simulink model "model"  (R2014a)
(part 8 of 8)

  T_26367884_110000_/LConn1 -- _CN_26391332_110000_CN_26367884_110000/RConn1
  T_26367884_110000_/LConn2 -- _CN_26391332_110000_CN_26367884_110000/RConn2
  _CN_26391332_110000_CN_26367884_110000/RConn3 -- T_26367884_110000_/LConn3 -- bus192/LConn1
  T_197245741_110000_/LConn1 -- _CN_197245741_110000_CN_128571463_110000/RConn1
  T_197245741_110000_/LConn2 -- _CN_197245741_110000_CN_128571463_110000/RConn2
  _CN_197245741_110000_CN_128571463_110000/RConn3 -- T_197245741_110000_/LConn3 -- bus193/LConn1
  _CN_117383986_110000_CN_153576520_110000/RConn1 -- T_153576520_110000_/LConn1 -- _CN_153576520_110000_CN_148596527_110000/RConn1
  _CN_117383986_110000_CN_153576520_110000/RConn2 -- T_153576520_110000_/LConn2 -- _CN_153576520_110000_CN_148596527_110000/RConn2
  _CN_117383986_110000_CN_153576520_110000/RConn3 -- T_153576520_110000_/LConn3 -- _CN_153576520_110000_CN_148596527_110000/RConn3 -- bus194/LConn1
  _CN_47317827_110000_CN_169899622_110000/LConn1 -- T_47317827_400000;110000_Keminmaan_sähköasema/RConn1 -- _CN_47317827_110000_CN_118766661_110000/RConn1 -- L_47317827/LConn1
  _CN_47317827_110000_CN_169899622_110000/LConn2 -- T_47317827_400000;110000_Keminmaan_sähköasema/RConn2 -- _CN_47317827_110000_CN_118766661_110000/RConn2 -- L_47317827/LConn2
  _CN_47317827_110000_CN_169899622_110000/LConn3 -- T_47317827_400000;110000_Keminmaan_sähköasema/RConn3 -- _CN_47317827_110000_CN_118766661_110000/RConn3 -- L_47317827/LConn3 -- bus195/LConn1
  _CN_47317827_110000_CN_169899622_110000/RConn1 -- T_169899622_220000;110000_/LConn1 -- _CN_169899622_110000_CN_169899620_20000/RConn1
  _CN_47317827_110000_CN_169899622_110000/RConn2 -- T_169899622_220000;110000_/LConn2 -- _CN_169899622_110000_CN_169899620_20000/RConn2
  _CN_47317827_110000_CN_169899622_110000/RConn3 -- T_169899622_220000;110000_/LConn3 -- _CN_169899622_110000_CN_169899620_20000/RConn3 -- bus196/LConn1
  _CN_137112425_110000_CN_132652863_110000/LConn1 -- T_137112425_110000_/LConn1 -- _CN_137112425_110000_CN_136355274_110000/LConn1
  _CN_137112425_110000_CN_132652863_110000/LConn2 -- T_137112425_110000_/LConn2 -- _CN_137112425_110000_CN_136355274_110000/LConn2
  _CN_137112425_110000_CN_132652863_110000/LConn3 -- T_137112425_110000_/LConn3 -- _CN_137112425_110000_CN_136355274_110000/LConn3 -- bus197/LConn1
  T_132652863__/LConn1 -- _CN_137112425_110000_CN_132652863_110000/RConn1
  T_132652863__/LConn2 -- _CN_137112425_110000_CN_132652863_110000/RConn2
  _CN_137112425_110000_CN_132652863_110000/RConn3 -- T_132652863__/LConn3 -- bus198/LConn1
  _CN_137112425_110000_CN_136355274_110000/RConn1 -- T_136355274_110000_/LConn1 -- _CN_136355274_110000_CN_136361669_110000/LConn1
  _CN_137112425_110000_CN_136355274_110000/RConn2 -- T_136355274_110000_/LConn2 -- _CN_136355274_110000_CN_136361669_110000/LConn2
  _CN_137112425_110000_CN_136355274_110000/RConn3 -- T_136355274_110000_/LConn3 -- _CN_136355274_110000_CN_136361669_110000/LConn3 -- bus199/LConn1
  T_211471223_110000_/LConn1 -- _CN_211471223_110000_CN_98613134_110000/LConn1
  T_211471223_110000_/LConn2 -- _CN_211471223_110000_CN_98613134_110000/LConn2
  _CN_211471223_110000_CN_98613134_110000/LConn3 -- T_211471223_110000_/LConn3 -- bus200/LConn1
  _CN_211471223_110000_CN_98613134_110000/RConn1 -- T_98613134_400000;110000_/RConn1 -- _CN_26501426_110000_CN_98613134_110000/RConn1 -- L_98613134/LConn1
  _CN_211471223_110000_CN_98613134_110000/RConn2 -- T_98613134_400000;110000_/RConn2 -- _CN_26501426_110000_CN_98613134_110000/RConn2 -- L_98613134/LConn2
  _CN_211471223_110000_CN_98613134_110000/RConn3 -- T_98613134_400000;110000_/RConn3 -- _CN_26501426_110000_CN_98613134_110000/RConn3 -- L_98613134/LConn3 -- bus201/LConn1
  T_129112047_110000_/LConn1 -- _CN_128463750_110000_CN_129112047_110000/RConn1
  T_129112047_110000_/LConn2 -- _CN_128463750_110000_CN_129112047_110000/RConn2
  _CN_128463750_110000_CN_129112047_110000/RConn3 -- T_129112047_110000_/LConn3 -- bus202/LConn1
  T_155899286_110000_/LConn1 -- _CN_128463750_110000_CN_155899286_110000/RConn1
  T_155899286_110000_/LConn2 -- _CN_128463750_110000_CN_155899286_110000/RConn2
  _CN_128463750_110000_CN_155899286_110000/RConn3 -- T_155899286_110000_/LConn3 -- bus203/LConn1
  T_94667682_110000_/LConn1 -- _CN_94667682_110000_CN_95184246_110000/LConn1
  T_94667682_110000_/LConn2 -- _CN_94667682_110000_CN_95184246_110000/LConn2
  _CN_94667682_110000_CN_95184246_110000/LConn3 -- T_94667682_110000_/LConn3 -- bus204/LConn1
  T_95184246_110000_/LConn1 -- _CN_94667682_110000_CN_95184246_110000/RConn1
  T_95184246_110000_/LConn2 -- _CN_94667682_110000_CN_95184246_110000/RConn2
  _CN_94667682_110000_CN_95184246_110000/RConn3 -- T_95184246_110000_/LConn3 -- bus205/LConn1
  T_142846911__/LConn1 -- _CN_142846911_110000_CN_142846913_110000/RConn1
  T_142846911__/LConn2 -- _CN_142846911_110000_CN_142846913_110000/RConn2
  _CN_142846911_110000_CN_142846913_110000/RConn3 -- T_142846911__/LConn3 -- bus206/LConn1
  T_200166363__/LConn1 -- _CN_200166363_110000_CN_173431812_110000/LConn1
  T_200166363__/LConn2 -- _CN_200166363_110000_CN_173431812_110000/LConn2
  _CN_200166363_110000_CN_173431812_110000/LConn3 -- T_200166363__/LConn3 -- bus207/LConn1
  _CN_200166363_110000_CN_173431812_110000/RConn1 -- T_173431812_220000;110000_/LConn1 -- _CN_173431812_110000_CN_285201507_110000/LConn1
  _CN_200166363_110000_CN_173431812_110000/RConn2 -- T_173431812_220000;110000_/LConn2 -- _CN_173431812_110000_CN_285201507_110000/LConn2
  _CN_200166363_110000_CN_173431812_110000/RConn3 -- T_173431812_220000;110000_/LConn3 -- _CN_173431812_110000_CN_285201507_110000/LConn3 -- bus208/LConn1
  _CN_400589797_110000_CN_61960767_110000/LConn1 -- T_400589797_110000_/LConn1 -- _CN_400589797_110000_CN_400588215_110000/LConn1 -- _CN_400589797_110000_CN_92656655_110000/LConn1 -- _CN_400589797_110000_CN_174266079_110000/LConn1
  _CN_400589797_110000_CN_61960767_110000/LConn2 -- T_400589797_110000_/LConn2 -- _CN_400589797_110000_CN_400588215_110000/LConn2 -- _CN_400589797_110000_CN_92656655_110000/LConn2 -- _CN_400589797_110000_CN_174266079_110000/LConn2
  _CN_400589797_110000_CN_61960767_110000/LConn3 -- T_400589797_110000_/LConn3 -- _CN_400589797_110000_CN_400588215_110000/LConn3 -- _CN_400589797_110000_CN_92656655_110000/LConn3 -- _CN_400589797_110000_CN_174266079_110000/LConn3 -- bus209/LConn1
  G_61960767_/RConn1 -- _CN_400589797_110000_CN_61960767_110000/RConn1
  G_61960767_/RConn2 -- _CN_400589797_110000_CN_61960767_110000/RConn2
  _CN_400589797_110000_CN_61960767_110000/RConn3 -- G_61960767_/RConn3 -- bus210/LConn1
  _CN_400589797_110000_CN_400588215_110000/RConn1 -- T_400588215_110000_/LConn1 -- _CN_400588215_110000_CN_400588216_110000/RConn1
  _CN_400589797_110000_CN_400588215_110000/RConn2 -- T_400588215_110000_/LConn2 -- _CN_400588215_110000_CN_400588216_110000/RConn2
  _CN_400589797_110000_CN_400588215_110000/RConn3 -- T_400588215_110000_/LConn3 -- _CN_400588215_110000_CN_400588216_110000/RConn3 -- bus211/LConn1
  _CN_400589797_110000_CN_92656655_110000/RConn1 -- T_92656655_110000_/LConn1 -- _CN_363802508_110000_CN_92656655_110000/LConn1
  _CN_400589797_110000_CN_92656655_110000/RConn2 -- T_92656655_110000_/LConn2 -- _CN_363802508_110000_CN_92656655_110000/LConn2
  _CN_400589797_110000_CN_92656655_110000/RConn3 -- T_92656655_110000_/LConn3 -- _CN_363802508_110000_CN_92656655_110000/LConn3 -- bus212/LConn1
  T_174266079__/LConn1 -- _CN_400589797_110000_CN_174266079_110000/RConn1
  T_174266079__/LConn2 -- _CN_400589797_110000_CN_174266079_110000/RConn2
  _CN_400589797_110000_CN_174266079_110000/RConn3 -- T_174266079__/LConn3 -- bus213/LConn1
  T_363802508_110000_/LConn1 -- _CN_363802508_110000_CN_92656655_110000/RConn1
  T_363802508_110000_/LConn2 -- _CN_363802508_110000_CN_92656655_110000/RConn2
  _CN_363802508_110000_CN_92656655_110000/RConn3 -- T_363802508_110000_/LConn3 -- bus214/LConn1
  _CN_96660466_110000_CN_98393115_110000/LConn1 -- T_96660466_400000;110000_/RConn1 -- L_96660466/LConn1
  _CN_96660466_110000_CN_98393115_110000/LConn2 -- T_96660466_400000;110000_/RConn2 -- L_96660466/LConn2
  _CN_96660466_110000_CN_98393115_110000/LConn3 -- T_96660466_400000;110000_/RConn3 -- L_96660466/LConn3 -- bus215/LConn1
  T_98393115_110000_/LConn1 -- _CN_96660466_110000_CN_98393115_110000/RConn1
  T_98393115_110000_/LConn2 -- _CN_96660466_110000_CN_98393115_110000/RConn2
  _CN_96660466_110000_CN_98393115_110000/RConn3 -- T_98393115_110000_/LConn3 -- bus216/LConn1
  T_391142388_220000;110000_/LConn1 -- _CN_391142388_110000_CN_391142037_110000/LConn1
  T_391142388_220000;110000_/LConn2 -- _CN_391142388_110000_CN_391142037_110000/LConn2
  _CN_391142388_110000_CN_391142037_110000/LConn3 -- T_391142388_220000;110000_/LConn3 -- bus217/LConn1
  T_391142037_110000_/LConn1 -- _CN_391142388_110000_CN_391142037_110000/RConn1
  T_391142037_110000_/LConn2 -- _CN_391142388_110000_CN_391142037_110000/RConn2
  _CN_391142388_110000_CN_391142037_110000/RConn3 -- T_391142037_110000_/LConn3 -- bus218/LConn1
  _CN_173431802_110000_CN_122703556_110000/LConn1 -- T_173431802_400000;110000_/RConn1 -- L_173431802/LConn1
  _CN_173431802_110000_CN_122703556_110000/LConn2 -- T_173431802_400000;110000_/RConn2 -- L_173431802/LConn2
  _CN_173431802_110000_CN_122703556_110000/LConn3 -- T_173431802_400000;110000_/RConn3 -- L_173431802/LConn3 -- bus219/LConn1
  T_122703556__/LConn1 -- _CN_173431802_110000_CN_122703556_110000/RConn1
  T_122703556__/LConn2 -- _CN_173431802_110000_CN_122703556_110000/RConn2
  _CN_173431802_110000_CN_122703556_110000/RConn3 -- T_122703556__/LConn3 -- bus220/LConn1
  T_285201507__/LConn1 -- _CN_173431812_110000_CN_285201507_110000/RConn1
  T_285201507__/LConn2 -- _CN_173431812_110000_CN_285201507_110000/RConn2
  _CN_173431812_110000_CN_285201507_110000/RConn3 -- T_285201507__/LConn3 -- bus221/LConn1
  _CN_235817994_110000_CN_89956002_110000/LConn1 -- T_235817994_110000_/LConn1 -- _CN_235817994_110000_CN_345672987_110000/LConn1 -- _CN_235817994_110000_CN_88020737_110000/LConn1 -- _CN_235817994_110000_CN_88020687_110000/LConn1
  _CN_235817994_110000_CN_89956002_110000/LConn2 -- T_235817994_110000_/LConn2 -- _CN_235817994_110000_CN_345672987_110000/LConn2 -- _CN_235817994_110000_CN_88020737_110000/LConn2 -- _CN_235817994_110000_CN_88020687_110000/LConn2
  _CN_235817994_110000_CN_89956002_110000/LConn3 -- T_235817994_110000_/LConn3 -- _CN_235817994_110000_CN_345672987_110000/LConn3 -- bus222/LConn1 -- _CN_235817994_110000_CN_88020737_110000/LConn3 -- _CN_235817994_110000_CN_88020687_110000/LConn3
  T_89956002_110000_/LConn1 -- _CN_235817994_110000_CN_89956002_110000/RConn1
  T_89956002_110000_/LConn2 -- _CN_235817994_110000_CN_89956002_110000/RConn2
  _CN_235817994_110000_CN_89956002_110000/RConn3 -- T_89956002_110000_/LConn3 -- bus223/LConn1
  T_88020737_110000_/LConn1 -- _CN_235817994_110000_CN_88020737_110000/RConn1
  T_88020737_110000_/LConn2 -- _CN_235817994_110000_CN_88020737_110000/RConn2
  _CN_235817994_110000_CN_88020737_110000/RConn3 -- T_88020737_110000_/LConn3 -- bus224/LConn1
  T_88020687_110000_/LConn1 -- _CN_235817994_110000_CN_88020687_110000/RConn1
  T_88020687_110000_/LConn2 -- _CN_235817994_110000_CN_88020687_110000/RConn2
  _CN_235817994_110000_CN_88020687_110000/RConn3 -- T_88020687_110000_/LConn3 -- bus225/LConn1
  _CN_235817994_110000_CN_345672987_110000/RConn1 -- T_345672987_110000_/LConn1 -- _CN_345672987_110000_CN_348349199_110000/LConn1
  _CN_235817994_110000_CN_345672987_110000/RConn2 -- T_345672987_110000_/LConn2 -- _CN_345672987_110000_CN_348349199_110000/LConn2
  _CN_235817994_110000_CN_345672987_110000/RConn3 -- T_345672987_110000_/LConn3 -- _CN_345672987_110000_CN_348349199_110000/LConn3 -- bus226/LConn1
  T_30483473__/LConn1 -- _CN_30483473_110000_CN_40101584_110000/RConn1
  T_30483473__/LConn2 -- _CN_30483473_110000_CN_40101584_110000/RConn2
  _CN_30483473_110000_CN_40101584_110000/RConn3 -- T_30483473__/LConn3 -- bus227/LConn1
  _CN_28785740_110000_CN_28820749_110000/RConn1 -- T_28820749_400000;110000_Länsisalmen_sähköasema/RConn1 -- L_28820749/LConn1
  _CN_28785740_110000_CN_28820749_110000/RConn2 -- T_28820749_400000;110000_Länsisalmen_sähköasema/RConn2 -- L_28820749/LConn2
  _CN_28785740_110000_CN_28820749_110000/RConn3 -- T_28820749_400000;110000_Länsisalmen_sähköasema/RConn3 -- L_28820749/LConn3 -- bus228/LConn1
  T_218734234__/LConn1 -- _CN_32910454_110000_CN_218734234_110000/RConn1
  T_218734234__/LConn2 -- _CN_32910454_110000_CN_218734234_110000/RConn2
  _CN_32910454_110000_CN_218734234_110000/RConn3 -- T_218734234__/LConn3 -- bus229/LConn1
  T_167705754_110000_/LConn1 -- _CN_32910454_110000_CN_167705754_110000/RConn1
  T_167705754_110000_/LConn2 -- _CN_32910454_110000_CN_167705754_110000/RConn2
  _CN_32910454_110000_CN_167705754_110000/RConn3 -- T_167705754_110000_/LConn3 -- bus230/LConn1
  T_122838157_110000_/LConn1 -- _CN_122838157_110000_CN_140227959_110000/LConn1
  T_122838157_110000_/LConn2 -- _CN_122838157_110000_CN_140227959_110000/LConn2
  _CN_122838157_110000_CN_140227959_110000/LConn3 -- T_122838157_110000_/LConn3 -- bus231/LConn1
  T_140227959_110000_/LConn1 -- _CN_122838157_110000_CN_140227959_110000/RConn1
  T_140227959_110000_/LConn2 -- _CN_122838157_110000_CN_140227959_110000/RConn2
  _CN_122838157_110000_CN_140227959_110000/RConn3 -- T_140227959_110000_/LConn3 -- bus232/LConn1
  T_167862173__/LConn1 -- _CN_98561229_110000_CN_167862173_110000/RConn1
  T_167862173__/LConn2 -- _CN_98561229_110000_CN_167862173_110000/RConn2
  _CN_98561229_110000_CN_167862173_110000/RConn3 -- T_167862173__/LConn3 -- bus233/LConn1
  T_345672928__/LConn1 -- _CN_345672928_110000_CN_40101584_110000/RConn1
  T_345672928__/LConn2 -- _CN_345672928_110000_CN_40101584_110000/RConn2
  _CN_345672928_110000_CN_40101584_110000/RConn3 -- T_345672928__/LConn3 -- bus234/LConn1
  _CN_348003562_110000_CN_238900636_110000/RConn1 -- T_348003562_400000;110000_/RConn1 -- _CN_348003562_110000_CN_219227505_110000/RConn1 -- L_348003562/LConn1
  _CN_348003562_110000_CN_238900636_110000/RConn2 -- T_348003562_400000;110000_/RConn2 -- _CN_348003562_110000_CN_219227505_110000/RConn2 -- L_348003562/LConn2
  _CN_348003562_110000_CN_238900636_110000/RConn3 -- T_348003562_400000;110000_/RConn3 -- _CN_348003562_110000_CN_219227505_110000/RConn3 -- L_348003562/LConn3 -- bus235/LConn1
  T_348349199_110000_/LConn1 -- _CN_345672987_110000_CN_348349199_110000/RConn1
  T_348349199_110000_/LConn2 -- _CN_345672987_110000_CN_348349199_110000/RConn2
  _CN_345672987_110000_CN_348349199_110000/RConn3 -- T_348349199_110000_/LConn3 -- bus236/LConn1
  T_162950429_110000_/LConn1 -- _CN_162950429_110000_CN_162690719_110000/LConn1
  T_162950429_110000_/LConn2 -- _CN_162950429_110000_CN_162690719_110000/LConn2
  _CN_162950429_110000_CN_162690719_110000/LConn3 -- T_162950429_110000_/LConn3 -- bus237/LConn1
  T_162690719_110000_/LConn1 -- _CN_162950429_110000_CN_162690719_110000/RConn1
  T_162690719_110000_/LConn2 -- _CN_162950429_110000_CN_162690719_110000/RConn2
  _CN_162950429_110000_CN_162690719_110000/RConn3 -- T_162690719_110000_/LConn3 -- bus238/LConn1
  T_252609822_110000_/LConn1 -- _CN_252609822_110000_CN_150204241_110000/RConn1
  T_252609822_110000_/LConn2 -- _CN_252609822_110000_CN_150204241_110000/RConn2
  _CN_252609822_110000_CN_150204241_110000/RConn3 -- T_252609822_110000_/LConn3 -- bus239/LConn1
  T_158219552_110000_/LConn1 -- _CN_158219552_110000_CN_158031219_110000/RConn1
  T_158219552_110000_/LConn2 -- _CN_158219552_110000_CN_158031219_110000/RConn2
  _CN_158219552_110000_CN_158031219_110000/RConn3 -- T_158219552_110000_/LConn3 -- bus240/LConn1
  T_149818659_110000_/LConn1 -- _CN_149818658_110000_CN_149818659_110000/RConn1
  T_149818659_110000_/LConn2 -- _CN_149818658_110000_CN_149818659_110000/RConn2
  _CN_149818658_110000_CN_149818659_110000/RConn3 -- T_149818659_110000_/LConn3 -- bus241/LConn1
  T_165373253_110000_/LConn1 -- _CN_165373253_110000_CN_154863454_110000/RConn1
  T_165373253_110000_/LConn2 -- _CN_165373253_110000_CN_154863454_110000/RConn2
  _CN_165373253_110000_CN_154863454_110000/RConn3 -- T_165373253_110000_/LConn3 -- bus242/LConn1
  T_130069830__/LConn1 -- _CN_130069830_110000_CN_130069831_110000/LConn1
  T_130069830__/LConn2 -- _CN_130069830_110000_CN_130069831_110000/LConn2
  _CN_130069830_110000_CN_130069831_110000/LConn3 -- T_130069830__/LConn3 -- bus243/LConn1
  T_130069831_110000_/LConn1 -- _CN_130069830_110000_CN_130069831_110000/RConn1
  T_130069831_110000_/LConn2 -- _CN_130069830_110000_CN_130069831_110000/RConn2
  _CN_130069830_110000_CN_130069831_110000/RConn3 -- T_130069831_110000_/LConn3 -- bus244/LConn1
  _CN_130069833_110000_CN_130069838_110000/RConn1 -- T_130069833_110000_/LConn1 -- _CN_130069833_110000_CN_136068907_110000/RConn1
  _CN_130069833_110000_CN_130069838_110000/RConn2 -- T_130069833_110000_/LConn2 -- _CN_130069833_110000_CN_136068907_110000/RConn2
  _CN_130069833_110000_CN_130069838_110000/RConn3 -- T_130069833_110000_/LConn3 -- _CN_130069833_110000_CN_136068907_110000/RConn3 -- bus245/LConn1
  _CN_159532385_110000_CN_108980081_110000/RConn1 -- T_159532385_400000;110000_/RConn1 -- L_159532385/LConn1
  _CN_159532385_110000_CN_108980081_110000/RConn2 -- T_159532385_400000;110000_/RConn2 -- L_159532385/LConn2
  _CN_159532385_110000_CN_108980081_110000/RConn3 -- T_159532385_400000;110000_/RConn3 -- L_159532385/LConn3 -- bus246/LConn1
  T_147699112__/LConn1 -- _CN_147699112_110000_CN_147699118_110000/LConn1
  T_147699112__/LConn2 -- _CN_147699112_110000_CN_147699118_110000/LConn2
  _CN_147699112_110000_CN_147699118_110000/LConn3 -- T_147699112__/LConn3 -- bus247/LConn1
  T_147699118_110000_/LConn1 -- _CN_147699112_110000_CN_147699118_110000/RConn1
  T_147699118_110000_/LConn2 -- _CN_147699112_110000_CN_147699118_110000/RConn2
  _CN_147699112_110000_CN_147699118_110000/RConn3 -- T_147699118_110000_/LConn3 -- bus248/LConn1
  _CN_98735006_110000_CN_400584163_110000/RConn1 -- T_98735006_400000;110000_/RConn1 -- L_98735006/LConn1
  _CN_98735006_110000_CN_400584163_110000/RConn2 -- T_98735006_400000;110000_/RConn2 -- L_98735006/LConn2
  _CN_98735006_110000_CN_400584163_110000/RConn3 -- T_98735006_400000;110000_/RConn3 -- L_98735006/LConn3 -- bus249/LConn1
  T_178234889_110000_/LConn1 -- _CN_26619335_110000_CN_178234889_110000/RConn1
  T_178234889_110000_/LConn2 -- _CN_26619335_110000_CN_178234889_110000/RConn2
  _CN_26619335_110000_CN_178234889_110000/RConn3 -- T_178234889_110000_/LConn3 -- bus250/LConn1
  T_178234890_110000_/LConn1 -- _CN_26619335_110000_CN_178234890_110000/RConn1
  T_178234890_110000_/LConn2 -- _CN_26619335_110000_CN_178234890_110000/RConn2
  _CN_26619335_110000_CN_178234890_110000/RConn3 -- T_178234890_110000_/LConn3 -- bus251/LConn1
  _CN_136355274_110000_CN_136361669_110000/RConn1 -- T_136361669_110000_/LConn1 -- _CN_136361666_110000_CN_136361669_110000/LConn1
  _CN_136355274_110000_CN_136361669_110000/RConn2 -- T_136361669_110000_/LConn2 -- _CN_136361666_110000_CN_136361669_110000/LConn2
  _CN_136355274_110000_CN_136361669_110000/RConn3 -- T_136361669_110000_/LConn3 -- _CN_136361666_110000_CN_136361669_110000/LConn3 -- bus252/LConn1
  T_159172094_110000_/LConn1 -- _CN_159172094_110000_CN_167040166_110000/RConn1
  T_159172094_110000_/LConn2 -- _CN_159172094_110000_CN_167040166_110000/RConn2
  _CN_159172094_110000_CN_167040166_110000/RConn3 -- T_159172094_110000_/LConn3 -- bus253/LConn1
  T_104410725__/LConn1 -- _CN_104410725_110000_CN_178181897_110000/LConn1
  T_104410725__/LConn2 -- _CN_104410725_110000_CN_178181897_110000/LConn2
  _CN_104410725_110000_CN_178181897_110000/LConn3 -- T_104410725__/LConn3 -- bus254/LConn1
  T_178181897_110000_/LConn1 -- _CN_104410725_110000_CN_178181897_110000/RConn1
  T_178181897_110000_/LConn2 -- _CN_104410725_110000_CN_178181897_110000/RConn2
  _CN_104410725_110000_CN_178181897_110000/RConn3 -- T_178181897_110000_/LConn3 -- bus255/LConn1
  _CN_198362738_110000_CN_198362740_110000/LConn1 -- T_198362738_110000_/LConn1 -- _CN_198362738_110000_CN_198362741_110000/LConn1
  _CN_198362738_110000_CN_198362740_110000/LConn2 -- T_198362738_110000_/LConn2 -- _CN_198362738_110000_CN_198362741_110000/LConn2
  _CN_198362738_110000_CN_198362740_110000/LConn3 -- T_198362738_110000_/LConn3 -- _CN_198362738_110000_CN_198362741_110000/LConn3 -- bus256/LConn1
  _CN_198362738_110000_CN_198362740_110000/RConn1 -- T_198362740_110000_/LConn1 -- _CN_198362740_110000_CN_198362741_110000/LConn1
  _CN_198362738_110000_CN_198362740_110000/RConn2 -- T_198362740_110000_/LConn2 -- _CN_198362740_110000_CN_198362741_110000/LConn2
  _CN_198362738_110000_CN_198362740_110000/RConn3 -- T_198362740_110000_/LConn3 -- _CN_198362740_110000_CN_198362741_110000/LConn3 -- bus257/LConn1
  _CN_198362738_110000_CN_198362741_110000/RConn1 -- T_198362741_110000_/LConn1 -- _CN_198362740_110000_CN_198362741_110000/RConn1
  _CN_198362738_110000_CN_198362741_110000/RConn2 -- T_198362741_110000_/LConn2 -- _CN_198362740_110000_CN_198362741_110000/RConn2
  _CN_198362738_110000_CN_198362741_110000/RConn3 -- T_198362741_110000_/LConn3 -- _CN_198362740_110000_CN_198362741_110000/RConn3 -- bus258/LConn1
  T_143511169_110000_/LConn1 -- _CN_143511169_110000_CN_143511171_110000/LConn1
  T_143511169_110000_/LConn2 -- _CN_143511169_110000_CN_143511171_110000/LConn2
  _CN_143511169_110000_CN_143511171_110000/LConn3 -- T_143511169_110000_/LConn3 -- bus259/LConn1
  T_143511171_110000_/LConn1 -- _CN_143511169_110000_CN_143511171_110000/RConn1
  T_143511171_110000_/LConn2 -- _CN_143511169_110000_CN_143511171_110000/RConn2
  _CN_143511169_110000_CN_143511171_110000/RConn3 -- T_143511171_110000_/LConn3 -- bus260/LConn1
  T_26330814_110000_/LConn1 -- _CN_26330814_110000_CN_53047221_110000/LConn1
  T_26330814_110000_/LConn2 -- _CN_26330814_110000_CN_53047221_110000/LConn2
  _CN_26330814_110000_CN_53047221_110000/LConn3 -- T_26330814_110000_/LConn3 -- bus261/LConn1
  T_53047221_110000_/LConn1 -- _CN_26330814_110000_CN_53047221_110000/RConn1
  T_53047221_110000_/LConn2 -- _CN_26330814_110000_CN_53047221_110000/RConn2
  _CN_26330814_110000_CN_53047221_110000/RConn3 -- T_53047221_110000_/LConn3 -- bus262/LConn1
  T_136361666_110000_/LConn1 -- _CN_136361666_110000_CN_136361669_110000/RConn1
  T_136361666_110000_/LConn2 -- _CN_136361666_110000_CN_136361669_110000/RConn2
  _CN_136361666_110000_CN_136361669_110000/RConn3 -- T_136361666_110000_/LConn3 -- bus263/LConn1
  T_87670542_110000_/LConn1 -- _CN_87670542_110000_CN_87670572_110000/RConn1
  T_87670542_110000_/LConn2 -- _CN_87670542_110000_CN_87670572_110000/RConn2
  _CN_87670542_110000_CN_87670572_110000/RConn3 -- T_87670542_110000_/LConn3 -- bus264/LConn1
  _CN_177676064_110000_CN_167176159_110000/LConn1 -- T_177676064__/LConn1 -- _CN_177676064_110000_CN_167184034_110000/LConn1
  _CN_177676064_110000_CN_167176159_110000/LConn2 -- T_177676064__/LConn2 -- _CN_177676064_110000_CN_167184034_110000/LConn2
  _CN_177676064_110000_CN_167176159_110000/LConn3 -- T_177676064__/LConn3 -- _CN_177676064_110000_CN_167184034_110000/LConn3 -- bus265/LConn1
  T_167176159_110000_/LConn1 -- _CN_177676064_110000_CN_167176159_110000/RConn1
  T_167176159_110000_/LConn2 -- _CN_177676064_110000_CN_167176159_110000/RConn2
  _CN_177676064_110000_CN_167176159_110000/RConn3 -- T_167176159_110000_/LConn3 -- bus266/LConn1
  T_167184034__/LConn1 -- _CN_177676064_110000_CN_167184034_110000/RConn1
  T_167184034__/LConn2 -- _CN_177676064_110000_CN_167184034_110000/RConn2
  _CN_177676064_110000_CN_167184034_110000/RConn3 -- T_167184034__/LConn3 -- bus267/LConn1
  T_400582573_110000_/LConn1 -- _CN_26501426_110000_CN_400582573_110000/RConn1
  T_400582573_110000_/LConn2 -- _CN_26501426_110000_CN_400582573_110000/RConn2
  _CN_26501426_110000_CN_400582573_110000/RConn3 -- T_400582573_110000_/LConn3 -- bus268/LConn1
  T_400582583_110000_/LConn1 -- _CN_26501426_110000_CN_400582583_110000/RConn1
  T_400582583_110000_/LConn2 -- _CN_26501426_110000_CN_400582583_110000/RConn2
  _CN_26501426_110000_CN_400582583_110000/RConn3 -- T_400582583_110000_/LConn3 -- bus269/LConn1
  _CN_391140226_400000_CN_149965739_400000/LConn1 -- T_391140226_400000_/LConn1 -- _CN_391140226_400000_CN_47317827_400000/LConn1 -- _CN_391140226_400000_CN_388655178_400000/LConn1
  _CN_391140226_400000_CN_149965739_400000/LConn2 -- T_391140226_400000_/LConn2 -- _CN_391140226_400000_CN_47317827_400000/LConn2 -- _CN_391140226_400000_CN_388655178_400000/LConn2
  _CN_391140226_400000_CN_149965739_400000/LConn3 -- T_391140226_400000_/LConn3 -- _CN_391140226_400000_CN_47317827_400000/LConn3 -- _CN_391140226_400000_CN_388655178_400000/LConn3 -- bus270/LConn1
  _CN_391140226_400000_CN_149965739_400000/RConn1 -- T_149965739_400000;110000_/LConn1 -- _CN_149965739_400000_CN_149965733_400000/LConn1 -- _CN_149965739_400000_CN_136068907_400000/LConn1
  _CN_391140226_400000_CN_149965739_400000/RConn2 -- T_149965739_400000;110000_/LConn2 -- _CN_149965739_400000_CN_149965733_400000/LConn2 -- _CN_149965739_400000_CN_136068907_400000/LConn2
  _CN_391140226_400000_CN_149965739_400000/RConn3 -- T_149965739_400000;110000_/LConn3 -- _CN_149965739_400000_CN_149965733_400000/LConn3 -- bus271/LConn1 -- _CN_149965739_400000_CN_136068907_400000/LConn3
  _CN_391140226_400000_CN_47317827_400000/RConn1 -- T_47317827_400000;110000_Keminmaan_sähköasema/LConn1 -- _CN_47317827_400000_CN_217032425_400000/LConn1 -- _CN_286955409_400000_CN_47317827_400000/LConn1
  _CN_391140226_400000_CN_47317827_400000/RConn2 -- T_47317827_400000;110000_Keminmaan_sähköasema/LConn2 -- _CN_47317827_400000_CN_217032425_400000/LConn2 -- _CN_286955409_400000_CN_47317827_400000/LConn2
  _CN_391140226_400000_CN_47317827_400000/RConn3 -- T_47317827_400000;110000_Keminmaan_sähköasema/LConn3 -- _CN_47317827_400000_CN_217032425_400000/LConn3 -- bus272/LConn1 -- _CN_286955409_400000_CN_47317827_400000/LConn3
  _CN_391140226_400000_CN_388655178_400000/RConn1 -- T_388655178_400000;220000;110000_/LConn1 -- _CN_388655178_400000_CN_388755097_400000/LConn1 -- _CN_286955409_400000_CN_388655178_400000/LConn1
  _CN_391140226_400000_CN_388655178_400000/RConn2 -- T_388655178_400000;220000;110000_/LConn2 -- _CN_388655178_400000_CN_388755097_400000/LConn2 -- _CN_286955409_400000_CN_388655178_400000/LConn2
  _CN_391140226_400000_CN_388655178_400000/RConn3 -- T_388655178_400000;220000;110000_/LConn3 -- _CN_388655178_400000_CN_388755097_400000/LConn3 -- bus273/LConn1 -- _CN_286955409_400000_CN_388655178_400000/LConn3
  _CN_149965739_400000_CN_136068907_400000/RConn1 -- T_136068907_400000;220000;110000_/LConn1 -- _CN_136068907_400000_CN_123462491_400000/LConn1 -- _CN_136068907_400000_CN_43143343_400000/LConn1 -- _CN_34623113_400000_CN_136068907_400000/LConn1
  _CN_149965739_400000_CN_136068907_400000/RConn2 -- T_136068907_400000;220000;110000_/LConn2 -- _CN_136068907_400000_CN_123462491_400000/LConn2 -- _CN_136068907_400000_CN_43143343_400000/LConn2 -- _CN_34623113_400000_CN_136068907_400000/LConn2
  _CN_149965739_400000_CN_136068907_400000/RConn3 -- T_136068907_400000;220000;110000_/LConn3 -- _CN_136068907_400000_CN_123462491_400000/LConn3 -- bus274/LConn1 -- _CN_136068907_400000_CN_43143343_400000/LConn3 -- _CN_34623113_400000_CN_136068907_400000/LConn3
  _CN_149965739_400000_CN_149965733_400000/RConn1 -- T_149965733_400000;220000_/LConn1 -- _CN_286955409_400000_CN_149965733_400000/LConn1 -- _CN_149965733_400000_CN_208979069_400000/LConn1
  _CN_149965739_400000_CN_149965733_400000/RConn2 -- T_149965733_400000;220000_/LConn2 -- _CN_286955409_400000_CN_149965733_400000/LConn2 -- _CN_149965733_400000_CN_208979069_400000/LConn2
  _CN_149965739_400000_CN_149965733_400000/RConn3 -- T_149965733_400000;220000_/LConn3 -- _CN_286955409_400000_CN_149965733_400000/LConn3 -- _CN_149965733_400000_CN_208979069_400000/LConn3 -- bus275/LConn1
  _CN_128463750_400000_CN_208979069_400000/LConn1 -- T_128463750_400000;110000_/LConn1 -- _CN_128463750_400000_CN_98736918_400000/LConn1
  _CN_128463750_400000_CN_208979069_400000/LConn2 -- T_128463750_400000;110000_/LConn2 -- _CN_128463750_400000_CN_98736918_400000/LConn2
  _CN_128463750_400000_CN_208979069_400000/LConn3 -- T_128463750_400000;110000_/LConn3 -- _CN_128463750_400000_CN_98736918_400000/LConn3 -- bus276/LConn1
  _CN_128463750_400000_CN_208979069_400000/RConn1 -- T_208979069_400000;110000_/LConn1 -- _CN_149965733_400000_CN_208979069_400000/RConn1
  _CN_128463750_400000_CN_208979069_400000/RConn2 -- T_208979069_400000;110000_/LConn2 -- _CN_149965733_400000_CN_208979069_400000/RConn2
  _CN_128463750_400000_CN_208979069_400000/RConn3 -- T_208979069_400000;110000_/LConn3 -- _CN_149965733_400000_CN_208979069_400000/RConn3 -- bus277/LConn1
  _CN_128463750_400000_CN_98736918_400000/RConn1 -- T_98736918_400000;110000_/LConn1 -- _CN_98736918_400000_CN_43143343_400000/LConn1
  _CN_128463750_400000_CN_98736918_400000/RConn2 -- T_98736918_400000;110000_/LConn2 -- _CN_98736918_400000_CN_43143343_400000/LConn2
  _CN_128463750_400000_CN_98736918_400000/RConn3 -- T_98736918_400000;110000_/LConn3 -- _CN_98736918_400000_CN_43143343_400000/LConn3 -- bus278/LConn1
  _CN_34623113_400000_CN_173431802_400000/LConn1 -- T_34623113_400000;110000_/LConn1 -- _CN_34623113_400000_CN_239242345_400000/LConn1 -- _CN_34623113_400000_CN_96660466_400000/LConn1 -- _CN_34623113_400000_CN_238856422_400000/LConn1 -- _CN_34623113_400000_CN_159532385_400000/LConn1 -- _CN_34623113_400000_CN_136068907_400000/RConn1
  _CN_34623113_400000_CN_173431802_400000/LConn2 -- T_34623113_400000;110000_/LConn2 -- _CN_34623113_400000_CN_239242345_400000/LConn2 -- _CN_34623113_400000_CN_96660466_400000/LConn2 -- _CN_34623113_400000_CN_238856422_400000/LConn2 -- _CN_34623113_400000_CN_159532385_400000/LConn2 -- _CN_34623113_400000_CN_136068907_400000/RConn2
  _CN_34623113_400000_CN_173431802_400000/LConn3 -- T_34623113_400000;110000_/LConn3 -- _CN_34623113_400000_CN_239242345_400000/LConn3 -- _CN_34623113_400000_CN_96660466_400000/LConn3 -- _CN_34623113_400000_CN_238856422_400000/LConn3 -- _CN_34623113_400000_CN_159532385_400000/LConn3 -- _CN_34623113_400000_CN_136068907_400000/RConn3 -- bus279/LConn1
  _CN_34623113_400000_CN_173431802_400000/RConn1 -- T_173431802_400000;110000_/LConn1 -- _CN_43143343_400000_CN_173431802_400000/LConn1
  _CN_34623113_400000_CN_173431802_400000/RConn2 -- T_173431802_400000;110000_/LConn2 -- _CN_43143343_400000_CN_173431802_400000/LConn2
  _CN_34623113_400000_CN_173431802_400000/RConn3 -- T_173431802_400000;110000_/LConn3 -- _CN_43143343_400000_CN_173431802_400000/LConn3 -- bus280/LConn1
  _CN_34623113_400000_CN_239242345_400000/RConn1 -- T_239242345_400000_/LConn1 -- _CN_98589905_400000_CN_239242345_400000/LConn1 -- _CN_98613134_400000_CN_239242345_400000/LConn1 -- _CN_98735006_400000_CN_239242345_400000/LConn1
  _CN_34623113_400000_CN_239242345_400000/RConn2 -- T_239242345_400000_/LConn2 -- _CN_98589905_400000_CN_239242345_400000/LConn2 -- _CN_98613134_400000_CN_239242345_400000/LConn2 -- _CN_98735006_400000_CN_239242345_400000/LConn2
  _CN_34623113_400000_CN_239242345_400000/RConn3 -- T_239242345_400000_/LConn3 -- _CN_98589905_400000_CN_239242345_400000/LConn3 -- bus281/LConn1 -- _CN_98613134_400000_CN_239242345_400000/LConn3 -- _CN_98735006_400000_CN_239242345_400000/LConn3
  T_96660466_400000;110000_/LConn1 -- _CN_34623113_400000_CN_96660466_400000/RConn1
  T_96660466_400000;110000_/LConn2 -- _CN_34623113_400000_CN_96660466_400000/RConn2
  _CN_34623113_400000_CN_96660466_400000/RConn3 -- T_96660466_400000;110000_/LConn3 -- bus282/LConn1
  _CN_34623113_400000_CN_238856422_400000/RConn1 -- T_238856422_400000;110000_/LConn1 -- _CN_348003562_400000_CN_238856422_400000/LConn1
  _CN_34623113_400000_CN_238856422_400000/RConn2 -- T_238856422_400000;110000_/LConn2 -- _CN_348003562_400000_CN_238856422_400000/LConn2
  _CN_34623113_400000_CN_238856422_400000/RConn3 -- T_238856422_400000;110000_/LConn3 -- _CN_348003562_400000_CN_238856422_400000/LConn3 -- bus283/LConn1
  _CN_34623113_400000_CN_159532385_400000/RConn1 -- T_159532385_400000;110000_/LConn1 -- _CN_26619335_400000_CN_159532385_400000/LConn1
  _CN_34623113_400000_CN_159532385_400000/RConn2 -- T_159532385_400000;110000_/LConn2 -- _CN_26619335_400000_CN_159532385_400000/LConn2
  _CN_34623113_400000_CN_159532385_400000/RConn3 -- T_159532385_400000;110000_/LConn3 -- _CN_26619335_400000_CN_159532385_400000/LConn3 -- bus284/LConn1
  _CN_28820749_400000_CN_25594007_400000/LConn1 -- T_28820749_400000;110000_Länsisalmen_sähköasema/LConn1 -- _CN_28820749_400000_CN_26619335_400000/LConn1 -- _CN_28820749_400000_CN_53047196_400000/LConn1 -- _CN_28820749_400000_CN_144832705_400000/LConn1
  _CN_28820749_400000_CN_25594007_400000/LConn2 -- T_28820749_400000;110000_Länsisalmen_sähköasema/LConn2 -- _CN_28820749_400000_CN_26619335_400000/LConn2 -- _CN_28820749_400000_CN_53047196_400000/LConn2 -- _CN_28820749_400000_CN_144832705_400000/LConn2
  _CN_28820749_400000_CN_25594007_400000/LConn3 -- T_28820749_400000;110000_Länsisalmen_sähköasema/LConn3 -- _CN_28820749_400000_CN_26619335_400000/LConn3 -- _CN_28820749_400000_CN_53047196_400000/LConn3 -- _CN_28820749_400000_CN_144832705_400000/LConn3 -- bus285/LConn1
  _CN_28820749_400000_CN_25594007_400000/RConn1 -- T_25594007_400000;110000_Tammiston_sähköasema/LConn1 -- _CN_25594007_400000_CN_98735006_400000/LConn1 -- Espoo_Tammisto_CN_25594007_400000_CN_27674611_400000/LConn1
  _CN_28820749_400000_CN_25594007_400000/RConn2 -- T_25594007_400000;110000_Tammiston_sähköasema/LConn2 -- _CN_25594007_400000_CN_98735006_400000/LConn2 -- Espoo_Tammisto_CN_25594007_400000_CN_27674611_400000/LConn2
  _CN_28820749_400000_CN_25594007_400000/RConn3 -- T_25594007_400000;110000_Tammiston_sähköasema/LConn3 -- _CN_25594007_400000_CN_98735006_400000/LConn3 -- Espoo_Tammisto_CN_25594007_400000_CN_27674611_400000/LConn3 -- bus286/LConn1
  _CN_28820749_400000_CN_26619335_400000/RConn1 -- T_26619335_400000;110000_/LConn1 -- _CN_26619335_400000_CN_159532385_400000/RConn1
  _CN_28820749_400000_CN_26619335_400000/RConn2 -- T_26619335_400000;110000_/LConn2 -- _CN_26619335_400000_CN_159532385_400000/RConn2
  _CN_28820749_400000_CN_26619335_400000/RConn3 -- T_26619335_400000;110000_/LConn3 -- _CN_26619335_400000_CN_159532385_400000/RConn3 -- bus287/LConn1
  _CN_28820749_400000_CN_53047196_400000/RConn1 -- T_53047196_400000_/LConn1 -- _CN_53047196_400000_CN_225399990_400000/LConn1 -- LO_KR_CN_53047196_400000_CN_35281467_400000/LConn1
  _CN_28820749_400000_CN_53047196_400000/RConn2 -- T_53047196_400000_/LConn2 -- _CN_53047196_400000_CN_225399990_400000/LConn2 -- LO_KR_CN_53047196_400000_CN_35281467_400000/LConn2
  _CN_28820749_400000_CN_53047196_400000/RConn3 -- T_53047196_400000_/LConn3 -- _CN_53047196_400000_CN_225399990_400000/LConn3 -- bus288/LConn1 -- LO_KR_CN_53047196_400000_CN_35281467_400000/LConn3
  _CN_28820749_400000_CN_144832705_400000/RConn1 -- T_144832705_400000;110000_/LConn1 -- KR_KM_CN_35281467_400000_CN_144832705_400000/LConn1
  _CN_28820749_400000_CN_144832705_400000/RConn2 -- T_144832705_400000;110000_/LConn2 -- KR_KM_CN_35281467_400000_CN_144832705_400000/LConn2
  _CN_28820749_400000_CN_144832705_400000/RConn3 -- T_144832705_400000;110000_/LConn3 -- KR_KM_CN_35281467_400000_CN_144832705_400000/LConn3 -- bus289/LConn1
  _CN_98613134_400000_CN_239242345_400000/RConn1 -- T_98613134_400000;110000_/LConn1 -- _CN_98613134_400000_CN_98589905_400000/LConn1 -- _CN_98613134_400000_CN_26501426_400000/LConn1 -- _CN_98613134_400000_CN_123462491_400000/LConn1
  _CN_98613134_400000_CN_239242345_400000/RConn2 -- T_98613134_400000;110000_/LConn2 -- _CN_98613134_400000_CN_98589905_400000/LConn2 -- _CN_98613134_400000_CN_26501426_400000/LConn2 -- _CN_98613134_400000_CN_123462491_400000/LConn2
  _CN_98613134_400000_CN_239242345_400000/RConn3 -- T_98613134_400000;110000_/LConn3 -- _CN_98613134_400000_CN_98589905_400000/LConn3 -- _CN_98613134_400000_CN_26501426_400000/LConn3 -- _CN_98613134_400000_CN_123462491_400000/LConn3 -- bus290/LConn1
  _CN_98613134_400000_CN_98589905_400000/RConn1 -- T_98589905_400000_/LConn1 -- _CN_98589905_400000_CN_26504079_400000/LConn1 -- _CN_98589905_400000_CN_239242345_400000/RConn1 -- _CN_98609844_400000_CN_98589905_400000/LConn1
  _CN_98613134_400000_CN_98589905_400000/RConn2 -- T_98589905_400000_/LConn2 -- _CN_98589905_400000_CN_26504079_400000/LConn2 -- _CN_98589905_400000_CN_239242345_400000/RConn2 -- _CN_98609844_400000_CN_98589905_400000/LConn2
  _CN_98613134_400000_CN_98589905_400000/RConn3 -- T_98589905_400000_/LConn3 -- _CN_98589905_400000_CN_26504079_400000/LConn3 -- bus291/LConn1 -- _CN_98589905_400000_CN_239242345_400000/RConn3 -- _CN_98609844_400000_CN_98589905_400000/LConn3
  _CN_98613134_400000_CN_26501426_400000/RConn1 -- T_26501426_400000;110000_/LConn1 -- _CN_151818544_400000_CN_26501426_400000/LConn1 -- HVDC_Fenno_Skan_CN_26501426_400000_CN_98554218_400000/LConn1
  _CN_98613134_400000_CN_26501426_400000/RConn2 -- T_26501426_400000;110000_/LConn2 -- _CN_151818544_400000_CN_26501426_400000/LConn2 -- HVDC_Fenno_Skan_CN_26501426_400000_CN_98554218_400000/LConn2
  _CN_98613134_400000_CN_26501426_400000/RConn3 -- T_26501426_400000;110000_/LConn3 -- _CN_151818544_400000_CN_26501426_400000/LConn3 -- HVDC_Fenno_Skan_CN_26501426_400000_CN_98554218_400000/LConn3 -- bus292/LConn1
  _CN_98613134_400000_CN_123462491_400000/RConn1 -- T_123462491_400000;110000_Empower/LConn1 -- Seinäjoki_Tuovila_CN_150209972_400000_CN_123462491_400000/LConn1 -- _CN_136068907_400000_CN_123462491_400000/RConn1
  _CN_98613134_400000_CN_123462491_400000/RConn2 -- T_123462491_400000;110000_Empower/LConn2 -- Seinäjoki_Tuovila_CN_150209972_400000_CN_123462491_400000/LConn2 -- _CN_136068907_400000_CN_123462491_400000/RConn2
  _CN_98613134_400000_CN_123462491_400000/RConn3 -- T_123462491_400000;110000_Empower/LConn3 -- Seinäjoki_Tuovila_CN_150209972_400000_CN_123462491_400000/LConn3 -- bus293/LConn1 -- _CN_136068907_400000_CN_123462491_400000/RConn3
  _CN_286955409_400000_CN_47317827_400000/RConn1 -- T_286955409_400000_Petäjäskoski/LConn1 -- _CN_286955409_400000_CN_388655178_400000/RConn1 -- _CN_286955409_400000_CN_149965733_400000/RConn1
  _CN_286955409_400000_CN_47317827_400000/RConn2 -- T_286955409_400000_Petäjäskoski/LConn2 -- _CN_286955409_400000_CN_388655178_400000/RConn2 -- _CN_286955409_400000_CN_149965733_400000/RConn2
  _CN_286955409_400000_CN_47317827_400000/RConn3 -- T_286955409_400000_Petäjäskoski/LConn3 -- _CN_286955409_400000_CN_388655178_400000/RConn3 -- bus294/LConn1 -- _CN_286955409_400000_CN_149965733_400000/RConn3
  _CN_98736918_400000_CN_43143343_400000/RConn1 -- T_43143343__/LConn1 -- _CN_136068907_400000_CN_43143343_400000/RConn1 -- _CN_43143343_400000_CN_173431802_400000/RConn1
  _CN_98736918_400000_CN_43143343_400000/RConn2 -- T_43143343__/LConn2 -- _CN_136068907_400000_CN_43143343_400000/RConn2 -- _CN_43143343_400000_CN_173431802_400000/RConn2
  _CN_98736918_400000_CN_43143343_400000/RConn3 -- T_43143343__/LConn3 -- _CN_136068907_400000_CN_43143343_400000/RConn3 -- _CN_43143343_400000_CN_173431802_400000/RConn3 -- bus295/LConn1
  _CN_25594007_400000_CN_98735006_400000/RConn1 -- T_98735006_400000;110000_/LConn1 -- _CN_98735006_400000_CN_239242345_400000/RConn1
  _CN_25594007_400000_CN_98735006_400000/RConn2 -- T_98735006_400000;110000_/LConn2 -- _CN_98735006_400000_CN_239242345_400000/RConn2
  _CN_25594007_400000_CN_98735006_400000/RConn3 -- T_98735006_400000;110000_/LConn3 -- _CN_98735006_400000_CN_239242345_400000/RConn3 -- bus296/LConn1
  Espoo_Tammisto_CN_25594007_400000_CN_27674611_400000/RConn1 -- T_27674611_400000;110000_/LConn1 -- _CN_348003562_400000_CN_27674611_400000/LConn1
  Espoo_Tammisto_CN_25594007_400000_CN_27674611_400000/RConn2 -- T_27674611_400000;110000_/LConn2 -- _CN_348003562_400000_CN_27674611_400000/LConn2
  Espoo_Tammisto_CN_25594007_400000_CN_27674611_400000/RConn3 -- T_27674611_400000;110000_/LConn3 -- _CN_348003562_400000_CN_27674611_400000/LConn3 -- bus297/LConn1
  LO_KR_CN_53047196_400000_CN_35281467_400000/RConn1 -- T_35281467_400000;110000_Korian_sähköasema/LConn1 -- KR_KM_CN_35281467_400000_CN_98561229_400000/LConn1 -- KR_KM_CN_35281467_400000_CN_144832705_400000/RConn1
  LO_KR_CN_53047196_400000_CN_35281467_400000/RConn2 -- T_35281467_400000;110000_Korian_sähköasema/LConn2 -- KR_KM_CN_35281467_400000_CN_98561229_400000/LConn2 -- KR_KM_CN_35281467_400000_CN_144832705_400000/RConn2
  LO_KR_CN_53047196_400000_CN_35281467_400000/RConn3 -- T_35281467_400000;110000_Korian_sähköasema/LConn3 -- KR_KM_CN_35281467_400000_CN_98561229_400000/LConn3 -- bus298/LConn1 -- KR_KM_CN_35281467_400000_CN_144832705_400000/RConn3
  G_225399990_Loviisan_ydinvoimalaitos/RConn1 -- _CN_53047196_400000_CN_225399990_400000/RConn1
  G_225399990_Loviisan_ydinvoimalaitos/RConn2 -- _CN_53047196_400000_CN_225399990_400000/RConn2
  _CN_53047196_400000_CN_225399990_400000/RConn3 -- G_225399990_Loviisan_ydinvoimalaitos/RConn3 -- bus299/LConn1
  T_348358044_400000;110000_/LConn1 -- _CN_348358044_400000_CN_98561229_400000/LConn1
  T_348358044_400000;110000_/LConn2 -- _CN_348358044_400000_CN_98561229_400000/LConn2
  _CN_348358044_400000_CN_98561229_400000/LConn3 -- T_348358044_400000;110000_/LConn3 -- bus300/LConn1
  _CN_348358044_400000_CN_98561229_400000/RConn1 -- T_98561229_400000;110000_/LConn1 -- KR_KM_CN_35281467_400000_CN_98561229_400000/RConn1
  _CN_348358044_400000_CN_98561229_400000/RConn2 -- T_98561229_400000;110000_/LConn2 -- KR_KM_CN_35281467_400000_CN_98561229_400000/RConn2
  _CN_348358044_400000_CN_98561229_400000/RConn3 -- T_98561229_400000;110000_/LConn3 -- KR_KM_CN_35281467_400000_CN_98561229_400000/RConn3 -- bus301/LConn1
  _CN_151818544_400000_CN_26501426_400000/RConn1 -- T_151818544_400000;110000_/LConn1 -- _CN_151818544_400000_CN_95392702_400000/LConn1 -- _CN_151818544_400000_CN_348003562_400000/LConn1
  _CN_151818544_400000_CN_26501426_400000/RConn2 -- T_151818544_400000;110000_/LConn2 -- _CN_151818544_400000_CN_95392702_400000/LConn2 -- _CN_151818544_400000_CN_348003562_400000/LConn2
  _CN_151818544_400000_CN_26501426_400000/RConn3 -- T_151818544_400000;110000_/LConn3 -- _CN_151818544_400000_CN_95392702_400000/LConn3 -- _CN_151818544_400000_CN_348003562_400000/LConn3 -- bus302/LConn1
  T_95392702_400000;110000_400kV_Salo/LConn1 -- _CN_151818544_400000_CN_95392702_400000/RConn1
  T_95392702_400000;110000_400kV_Salo/LConn2 -- _CN_151818544_400000_CN_95392702_400000/RConn2
  _CN_151818544_400000_CN_95392702_400000/RConn3 -- T_95392702_400000;110000_400kV_Salo/LConn3 -- bus303/LConn1
  _CN_151818544_400000_CN_348003562_400000/RConn1 -- T_348003562_400000;110000_/LConn1 -- _CN_348003562_400000_CN_27674611_400000/RConn1 -- _CN_348003562_400000_CN_238856422_400000/RConn1 -- _CN_348003562_400000_CN_238900636_110000/RConn1
  _CN_151818544_400000_CN_348003562_400000/RConn2 -- T_348003562_400000;110000_/LConn2 -- _CN_348003562_400000_CN_27674611_400000/RConn2 -- _CN_348003562_400000_CN_238856422_400000/RConn2 -- _CN_348003562_400000_CN_238900636_110000/RConn2
  _CN_151818544_400000_CN_348003562_400000/RConn3 -- T_348003562_400000;110000_/LConn3 -- _CN_348003562_400000_CN_27674611_400000/RConn3 -- _CN_348003562_400000_CN_238856422_400000/RConn3 -- bus304/LConn1 -- _CN_348003562_400000_CN_238900636_110000/RConn3
  T_98554218__/LConn1 -- HVDC_Fenno_Skan_CN_26501426_400000_CN_98554218_400000/RConn1
  T_98554218__/LConn2 -- HVDC_Fenno_Skan_CN_26501426_400000_CN_98554218_400000/RConn2
  HVDC_Fenno_Skan_CN_26501426_400000_CN_98554218_400000/RConn3 -- T_98554218__/LConn3 -- bus305/LConn1
  T_98609844_400000_/LConn1 -- _CN_98609844_400000_CN_98589905_400000/RConn1
  T_98609844_400000_/LConn2 -- _CN_98609844_400000_CN_98589905_400000/RConn2
  _CN_98609844_400000_CN_98589905_400000/RConn3 -- T_98609844_400000_/LConn3 -- bus306/LConn1
  T_150209972_400000;110000_Tuovila/LConn1 -- Seinäjoki_Tuovila_CN_150209972_400000_CN_123462491_400000/RConn1
  T_150209972_400000;110000_Tuovila/LConn2 -- Seinäjoki_Tuovila_CN_150209972_400000_CN_123462491_400000/RConn2
  Seinäjoki_Tuovila_CN_150209972_400000_CN_123462491_400000/RConn3 -- T_150209972_400000;110000_Tuovila/LConn3 -- bus307/LConn1
  T_217032425_400000_/LConn1 -- _CN_47317827_400000_CN_217032425_400000/RConn1
  T_217032425_400000_/LConn2 -- _CN_47317827_400000_CN_217032425_400000/RConn2
  _CN_47317827_400000_CN_217032425_400000/RConn3 -- T_217032425_400000_/LConn3 -- bus308/LConn1
  G_388755097_/RConn1 -- _CN_388655178_400000_CN_388755097_400000/RConn1
  G_388755097_/RConn2 -- _CN_388655178_400000_CN_388755097_400000/RConn2
  _CN_388655178_400000_CN_388755097_400000/RConn3 -- G_388755097_/RConn3 -- bus309/LConn1
  G_26504079_Olkiluodon_ydinvoimala/RConn1 -- _CN_98589905_400000_CN_26504079_400000/RConn1
  G_26504079_Olkiluodon_ydinvoimala/RConn2 -- _CN_98589905_400000_CN_26504079_400000/RConn2
  _CN_98589905_400000_CN_26504079_400000/RConn3 -- G_26504079_Olkiluodon_ydinvoimala/RConn3 -- bus310/LConn1
  T_88379010_220000;110000_/RConn1 -- L_88379010/LConn1
  T_88379010_220000;110000_/RConn2 -- L_88379010/LConn2
  L_88379010/LConn3 -- T_88379010_220000;110000_/RConn3 -- bus311/LConn1
  T_33691043_220000;110000_/RConn1 -- L_33691043/LConn1
  T_33691043_220000;110000_/RConn2 -- L_33691043/LConn2
  L_33691043/LConn3 -- T_33691043_220000;110000_/RConn3 -- bus312/LConn1
  T_150282502_220000_/RConn1 -- L_150282502/LConn1
  T_150282502_220000_/RConn2 -- L_150282502/LConn2
  L_150282502/LConn3 -- T_150282502_220000_/RConn3 -- bus313/LConn1
  T_314853393_220000;110000_/RConn1 -- L_314853393/LConn1
  T_314853393_220000;110000_/RConn2 -- L_314853393/LConn2
  L_314853393/LConn3 -- T_314853393_220000;110000_/RConn3 -- bus314/LConn1
  T_391145068_220000;110000_/RConn1 -- L_391145068/LConn1
  T_391145068_220000;110000_/RConn2 -- L_391145068/LConn2
  L_391145068/LConn3 -- T_391145068_220000;110000_/RConn3 -- bus315/LConn1
  T_55609623_220000;110000_/RConn1 -- L_55609623/LConn1
  T_55609623_220000;110000_/RConn2 -- L_55609623/LConn2
  L_55609623/LConn3 -- T_55609623_220000;110000_/RConn3 -- bus316/LConn1
  T_391142034_220000_/RConn1 -- L_391142034/LConn1
  T_391142034_220000_/RConn2 -- L_391142034/LConn2
  L_391142034/LConn3 -- T_391142034_220000_/RConn3 -- bus317/LConn1
  T_286955411_220000_/RConn1 -- L_286955411/LConn1
  T_286955411_220000_/RConn2 -- L_286955411/LConn2
  L_286955411/LConn3 -- T_286955411_220000_/RConn3 -- bus318/LConn1
  T_388832477_220000_Ossauskoski/RConn1 -- L_388832477/LConn1
  T_388832477_220000_Ossauskoski/RConn2 -- L_388832477/LConn2
  L_388832477/LConn3 -- T_388832477_220000_Ossauskoski/RConn3 -- bus319/LConn1
  T_400567451_220000_/RConn1 -- L_400567451/LConn1
  T_400567451_220000_/RConn2 -- L_400567451/LConn2
  L_400567451/LConn3 -- T_400567451_220000_/RConn3 -- bus320/LConn1
  T_149965738_220000_/RConn1 -- L_149965738/LConn1
  T_149965738_220000_/RConn2 -- L_149965738/LConn2
  L_149965738/LConn3 -- T_149965738_220000_/RConn3 -- bus321/LConn1
  T_169057271_220000_/RConn1 -- L_169057271/LConn1
  T_169057271_220000_/RConn2 -- L_169057271/LConn2
  L_169057271/LConn3 -- T_169057271_220000_/RConn3 -- bus322/LConn1
  T_169057270_220000_/RConn1 -- L_169057270/LConn1
  T_169057270_220000_/RConn2 -- L_169057270/LConn2
  L_169057270/LConn3 -- T_169057270_220000_/RConn3 -- bus323/LConn1
  T_75612161_110000_/RConn1 -- L_75612161/LConn1
  T_75612161_110000_/RConn2 -- L_75612161/LConn2
  L_75612161/LConn3 -- T_75612161_110000_/RConn3 -- bus324/LConn1
  T_28604436_110000_Suvilahti/RConn1 -- L_28604436/LConn1
  T_28604436_110000_Suvilahti/RConn2 -- L_28604436/LConn2
  L_28604436/LConn3 -- T_28604436_110000_Suvilahti/RConn3 -- bus325/LConn1
  T_6268760_110000_Herttoniemi/RConn1 -- L_6268760/LConn1
  T_6268760_110000_Herttoniemi/RConn2 -- L_6268760/LConn2
  L_6268760/LConn3 -- T_6268760_110000_Herttoniemi/RConn3 -- bus326/LConn1
  T_232208451__/RConn1 -- L_232208451/LConn1
  T_232208451__/RConn2 -- L_232208451/LConn2
  L_232208451/LConn3 -- T_232208451__/RConn3 -- bus327/LConn1
  T_187430983_110000_/RConn1 -- L_187430983/LConn1
  T_187430983_110000_/RConn2 -- L_187430983/LConn2
  L_187430983/LConn3 -- T_187430983_110000_/RConn3 -- bus328/LConn1
  T_209207437_110000_/RConn1 -- L_209207437/LConn1
  T_209207437_110000_/RConn2 -- L_209207437/LConn2
  L_209207437/LConn3 -- T_209207437_110000_/RConn3 -- bus329/LConn1
  T_187428237_110000_/RConn1 -- L_187428237/LConn1
  T_187428237_110000_/RConn2 -- L_187428237/LConn2
  L_187428237/LConn3 -- T_187428237_110000_/RConn3 -- bus330/LConn1
  T_128571465__/RConn1 -- L_128571465/LConn1
  T_128571465__/RConn2 -- L_128571465/LConn2
  L_128571465/LConn3 -- T_128571465__/RConn3 -- bus331/LConn1
  T_128571463_110000_/RConn1 -- L_128571463/LConn1
  T_128571463_110000_/RConn2 -- L_128571463/LConn2
  L_128571463/LConn3 -- T_128571463_110000_/RConn3 -- bus332/LConn1
  T_42594389_110000_Kangasvuoren_sähköasema/RConn1 -- L_42594389/LConn1
  T_42594389_110000_Kangasvuoren_sähköasema/RConn2 -- L_42594389/LConn2
  L_42594389/LConn3 -- T_42594389_110000_Kangasvuoren_sähköasema/RConn3 -- bus333/LConn1
  T_285480163__/RConn1 -- L_285480163/LConn1
  T_285480163__/RConn2 -- L_285480163/LConn2
  L_285480163/LConn3 -- T_285480163__/RConn3 -- bus334/LConn1
  T_87670572_110000_/RConn1 -- L_87670572/LConn1
  T_87670572_110000_/RConn2 -- L_87670572/LConn2
  L_87670572/LConn3 -- T_87670572_110000_/RConn3 -- bus335/LConn1
  T_59014204__Hämeenlahden_sähköasema/RConn1 -- L_59014204/LConn1
  T_59014204__Hämeenlahden_sähköasema/RConn2 -- L_59014204/LConn2
  L_59014204/LConn3 -- T_59014204__Hämeenlahden_sähköasema/RConn3 -- bus336/LConn1
  T_151998558_110000_/RConn1 -- L_151998558/LConn1
  T_151998558_110000_/RConn2 -- L_151998558/LConn2
  L_151998558/LConn3 -- T_151998558_110000_/RConn3 -- bus337/LConn1
  T_159153725__/RConn1 -- L_159153725/LConn1
  T_159153725__/RConn2 -- L_159153725/LConn2
  L_159153725/LConn3 -- T_159153725__/RConn3 -- bus338/LConn1
  T_27175012__/RConn1 -- L_27175012/LConn1
  T_27175012__/RConn2 -- L_27175012/LConn2
  L_27175012/LConn3 -- T_27175012__/RConn3 -- bus339/LConn1
  T_108980081_110000_/RConn1 -- L_108980081/LConn1
  T_108980081_110000_/RConn2 -- L_108980081/LConn2
  L_108980081/LConn3 -- T_108980081_110000_/RConn3 -- bus340/LConn1
  T_178370665__/RConn1 -- L_178370665/LConn1
  T_178370665__/RConn2 -- L_178370665/LConn2
  L_178370665/LConn3 -- T_178370665__/RConn3 -- bus341/LConn1
  T_26358836_110000_/RConn1 -- L_26358836/LConn1
  T_26358836_110000_/RConn2 -- L_26358836/LConn2
  L_26358836/LConn3 -- T_26358836_110000_/RConn3 -- bus342/LConn1
  T_29421693_110000_/RConn1 -- L_29421693/LConn1
  T_29421693_110000_/RConn2 -- L_29421693/LConn2
  L_29421693/LConn3 -- T_29421693_110000_/RConn3 -- bus343/LConn1
  T_169259235__/RConn1 -- L_169259235/LConn1
  T_169259235__/RConn2 -- L_169259235/LConn2
  L_169259235/LConn3 -- T_169259235__/RConn3 -- bus344/LConn1
  T_130331348_110000_/RConn1 -- L_130331348/LConn1
  T_130331348_110000_/RConn2 -- L_130331348/LConn2
  L_130331348/LConn3 -- T_130331348_110000_/RConn3 -- bus345/LConn1
  T_352399506_110000_/RConn1 -- L_352399506/LConn1
  T_352399506_110000_/RConn2 -- L_352399506/LConn2
  L_352399506/LConn3 -- T_352399506_110000_/RConn3 -- bus346/LConn1
  T_136370546_110000_/RConn1 -- L_136370546/LConn1
  T_136370546_110000_/RConn2 -- L_136370546/LConn2
  L_136370546/LConn3 -- T_136370546_110000_/RConn3 -- bus347/LConn1
  T_28502182_110000_/RConn1 -- L_28502182/LConn1
  T_28502182_110000_/RConn2 -- L_28502182/LConn2
  L_28502182/LConn3 -- T_28502182_110000_/RConn3 -- bus348/LConn1
  T_31127270_110000_/RConn1 -- L_31127270/LConn1
  T_31127270_110000_/RConn2 -- L_31127270/LConn2
  L_31127270/LConn3 -- T_31127270_110000_/RConn3 -- bus349/LConn1
  T_28785740_110000_/RConn1 -- L_28785740/LConn1
  T_28785740_110000_/RConn2 -- L_28785740/LConn2
  L_28785740/LConn3 -- T_28785740_110000_/RConn3 -- bus350/LConn1
  T_26331359_110000_/RConn1 -- L_26331359/LConn1
  T_26331359_110000_/RConn2 -- L_26331359/LConn2
  L_26331359/LConn3 -- T_26331359_110000_/RConn3 -- bus351/LConn1
  T_25597544__Kannelmaki/RConn1 -- L_25597544/LConn1
  T_25597544__Kannelmaki/RConn2 -- L_25597544/LConn2
  L_25597544/LConn3 -- T_25597544__Kannelmaki/RConn3 -- bus352/LConn1
  T_155555327_110000_Myyrmäen_sähköasema/RConn1 -- L_155555327/LConn1
  T_155555327_110000_Myyrmäen_sähköasema/RConn2 -- L_155555327/LConn2
  L_155555327/LConn3 -- T_155555327_110000_Myyrmäen_sähköasema/RConn3 -- bus353/LConn1
  T_25598183__/RConn1 -- L_25598183/LConn1
  T_25598183__/RConn2 -- L_25598183/LConn2
  L_25598183/LConn3 -- T_25598183__/RConn3 -- bus354/LConn1
  T_177308630_110000_/RConn1 -- L_177308630/LConn1
  T_177308630_110000_/RConn2 -- L_177308630/LConn2
  L_177308630/LConn3 -- T_177308630_110000_/RConn3 -- bus355/LConn1
  T_25593756_110000_Viikki/RConn1 -- L_25593756/LConn1
  T_25593756_110000_Viikki/RConn2 -- L_25593756/LConn2
  L_25593756/LConn3 -- T_25593756_110000_Viikki/RConn3 -- bus356/LConn1
  T_136363036_110000_/RConn1 -- L_136363036/LConn1
  T_136363036_110000_/RConn2 -- L_136363036/LConn2
  L_136363036/LConn3 -- T_136363036_110000_/RConn3 -- bus357/LConn1
  T_152333104_110000_/RConn1 -- L_152333104/LConn1
  T_152333104_110000_/RConn2 -- L_152333104/LConn2
  L_152333104/LConn3 -- T_152333104_110000_/RConn3 -- bus358/LConn1
  T_130069838__/RConn1 -- L_130069838/LConn1
  T_130069838__/RConn2 -- L_130069838/LConn2
  L_130069838/LConn3 -- T_130069838__/RConn3 -- bus359/LConn1
  T_145567915_110000_/RConn1 -- L_145567915/LConn1
  T_145567915_110000_/RConn2 -- L_145567915/LConn2
  L_145567915/LConn3 -- T_145567915_110000_/RConn3 -- bus360/LConn1
  T_136909652__/RConn1 -- L_136909652/LConn1
  T_136909652__/RConn2 -- L_136909652/LConn2
  L_136909652/LConn3 -- T_136909652__/RConn3 -- bus361/LConn1
  T_186886932_110000_/RConn1 -- L_186886932/LConn1
  T_186886932_110000_/RConn2 -- L_186886932/LConn2
  L_186886932/LConn3 -- T_186886932_110000_/RConn3 -- bus362/LConn1
  T_128255187_110000_/RConn1 -- L_128255187/LConn1
  T_128255187_110000_/RConn2 -- L_128255187/LConn2
  L_128255187/LConn3 -- T_128255187_110000_/RConn3 -- bus363/LConn1
  T_397651041__/RConn1 -- L_397651041/LConn1
  T_397651041__/RConn2 -- L_397651041/LConn2
  L_397651041/LConn3 -- T_397651041__/RConn3 -- bus364/LConn1
  T_375670534_110000_/RConn1 -- L_375670534/LConn1
  T_375670534_110000_/RConn2 -- L_375670534/LConn2
  L_375670534/LConn3 -- T_375670534_110000_/RConn3 -- bus365/LConn1
  T_169224396__Pyhäveden_sähköasema/RConn1 -- L_169224396/LConn1
  T_169224396__Pyhäveden_sähköasema/RConn2 -- L_169224396/LConn2
  L_169224396/LConn3 -- T_169224396__Pyhäveden_sähköasema/RConn3 -- bus366/LConn1
  T_242586528_110000_/RConn1 -- L_242586528/LConn1
  T_242586528_110000_/RConn2 -- L_242586528/LConn2
  L_242586528/LConn3 -- T_242586528_110000_/RConn3 -- bus367/LConn1
  T_43140269__Vuosaaren_sähköasema/RConn1 -- L_43140269/LConn1
  T_43140269__Vuosaaren_sähköasema/RConn2 -- L_43140269/LConn2
  L_43140269/LConn3 -- T_43140269__Vuosaaren_sähköasema/RConn3 -- bus368/LConn1
  T_87697632__/RConn1 -- L_87697632/LConn1
  T_87697632__/RConn2 -- L_87697632/LConn2
  L_87697632/LConn3 -- T_87697632__/RConn3 -- bus369/LConn1
  T_363802509_110000_/RConn1 -- L_363802509/LConn1
  T_363802509_110000_/RConn2 -- L_363802509/LConn2
  L_363802509/LConn3 -- T_363802509_110000_/RConn3 -- bus370/LConn1
  T_219227505__/RConn1 -- L_219227505/LConn1
  T_219227505__/RConn2 -- L_219227505/LConn2
  L_219227505/LConn3 -- T_219227505__/RConn3 -- bus371/LConn1
  T_28085992__/RConn1 -- L_28085992/LConn1
  T_28085992__/RConn2 -- L_28085992/LConn2
  L_28085992/LConn3 -- T_28085992__/RConn3 -- bus372/LConn1
  T_299874537__/RConn1 -- L_299874537/LConn1
  T_299874537__/RConn2 -- L_299874537/LConn2
  L_299874537/LConn3 -- T_299874537__/RConn3 -- bus373/LConn1
  T_143778041_110000_/RConn1 -- L_143778041/LConn1
  T_143778041_110000_/RConn2 -- L_143778041/LConn2
  L_143778041/LConn3 -- T_143778041_110000_/RConn3 -- bus374/LConn1
  T_149954884_110000_/RConn1 -- L_149954884/LConn1
  T_149954884_110000_/RConn2 -- L_149954884/LConn2
  L_149954884/LConn3 -- T_149954884_110000_/RConn3 -- bus375/LConn1
  T_152740092_110000_/RConn1 -- L_152740092/LConn1
  T_152740092_110000_/RConn2 -- L_152740092/LConn2
  L_152740092/LConn3 -- T_152740092_110000_/RConn3 -- bus376/LConn1
  T_149818658_110000_/RConn1 -- L_149818658/LConn1
  T_149818658_110000_/RConn2 -- L_149818658/LConn2
  L_149818658/LConn3 -- T_149818658_110000_/RConn3 -- bus377/LConn1
  T_159693074__/RConn1 -- L_159693074/LConn1
  T_159693074__/RConn2 -- L_159693074/LConn2
  L_159693074/LConn3 -- T_159693074__/RConn3 -- bus378/LConn1
  T_152181013_110000_/RConn1 -- L_152181013/LConn1
  T_152181013_110000_/RConn2 -- L_152181013/LConn2
  L_152181013/LConn3 -- T_152181013_110000_/RConn3 -- bus379/LConn1
  T_157677847_110000_/RConn1 -- L_157677847/LConn1
  T_157677847_110000_/RConn2 -- L_157677847/LConn2
  L_157677847/LConn3 -- T_157677847_110000_/RConn3 -- bus380/LConn1
  T_302047780_110000_/RConn1 -- L_302047780/LConn1
  T_302047780_110000_/RConn2 -- L_302047780/LConn2
  L_302047780/LConn3 -- T_302047780_110000_/RConn3 -- bus381/LConn1
  T_57845262_110000_/RConn1 -- L_57845262/LConn1
  T_57845262_110000_/RConn2 -- L_57845262/LConn2
  L_57845262/LConn3 -- T_57845262_110000_/RConn3 -- bus382/LConn1
  T_119141766__/RConn1 -- L_119141766/LConn1
  T_119141766__/RConn2 -- L_119141766/LConn2
  L_119141766/LConn3 -- T_119141766__/RConn3 -- bus383/LConn1
  T_399014185_110000_/RConn1 -- L_399014185/LConn1
  T_399014185_110000_/RConn2 -- L_399014185/LConn2
  L_399014185/LConn3 -- T_399014185_110000_/RConn3 -- bus384/LConn1
  T_168877874_110000_/RConn1 -- L_168877874/LConn1
  T_168877874_110000_/RConn2 -- L_168877874/LConn2
  L_168877874/LConn3 -- T_168877874_110000_/RConn3 -- bus385/LConn1
  T_400584163__/RConn1 -- L_400584163/LConn1
  T_400584163__/RConn2 -- L_400584163/LConn2
  L_400584163/LConn3 -- T_400584163__/RConn3 -- bus386/LConn1
  T_151818564_110000_/RConn1 -- L_151818564/LConn1
  T_151818564_110000_/RConn2 -- L_151818564/LConn2
  L_151818564/LConn3 -- T_151818564_110000_/RConn3 -- bus387/LConn1
  T_51420019_110000_/RConn1 -- L_51420019/LConn1
  T_51420019_110000_/RConn2 -- L_51420019/LConn2
  L_51420019/LConn3 -- T_51420019_110000_/RConn3 -- bus388/LConn1
  T_400588216_110000_/RConn1 -- L_400588216/LConn1
  T_400588216_110000_/RConn2 -- L_400588216/LConn2
  L_400588216/LConn3 -- T_400588216_110000_/RConn3 -- bus389/LConn1
  T_143419698_110000;25000_Lamminpää_SA/RConn1 -- L_143419698/LConn1
  T_143419698_110000;25000_Lamminpää_SA/RConn2 -- L_143419698/LConn2
  L_143419698/LConn3 -- T_143419698_110000;25000_Lamminpää_SA/RConn3 -- bus390/LConn1
  T_142846914_110000_/RConn1 -- L_142846914/LConn1
  T_142846914_110000_/RConn2 -- L_142846914/LConn2
  L_142846914/LConn3 -- T_142846914_110000_/RConn3 -- bus391/LConn1
  T_161022271_110000_/RConn1 -- L_161022271/LConn1
  T_161022271_110000_/RConn2 -- L_161022271/LConn2
  L_161022271/LConn3 -- T_161022271_110000_/RConn3 -- bus392/LConn1
  T_161022023__/RConn1 -- L_161022023/LConn1
  T_161022023__/RConn2 -- L_161022023/LConn2
  L_161022023/LConn3 -- T_161022023__/RConn3 -- bus393/LConn1
  T_154863454_110000_/RConn1 -- L_154863454/LConn1
  T_154863454_110000_/RConn2 -- L_154863454/LConn2
  L_154863454/LConn3 -- T_154863454_110000_/RConn3 -- bus394/LConn1
  T_151818569_110000_/RConn1 -- L_151818569/LConn1
  T_151818569_110000_/RConn2 -- L_151818569/LConn2
  L_151818569/LConn3 -- T_151818569_110000_/RConn3 -- bus395/LConn1
  T_320110941_110000;25000_Rännäri_SA/RConn1 -- L_320110941/LConn1
  T_320110941_110000;25000_Rännäri_SA/RConn2 -- L_320110941/LConn2
  L_320110941/LConn3 -- T_320110941_110000;25000_Rännäri_SA/RConn3 -- bus396/LConn1
  T_151206413_110000;25000_Pahaneva_SA/RConn1 -- L_151206413/LConn1
  T_151206413_110000;25000_Pahaneva_SA/RConn2 -- L_151206413/LConn2
  L_151206413/LConn3 -- T_151206413_110000;25000_Pahaneva_SA/RConn3 -- bus397/LConn1
  T_142846913_110000;25000_Sisättö_SA/RConn1 -- L_142846913/LConn1
  T_142846913_110000;25000_Sisättö_SA/RConn2 -- L_142846913/LConn2
  L_142846913/LConn3 -- T_142846913_110000;25000_Sisättö_SA/RConn3 -- bus398/LConn1
  T_159825638_110000_/RConn1 -- L_159825638/LConn1
  T_159825638_110000_/RConn2 -- L_159825638/LConn2
  L_159825638/LConn3 -- T_159825638_110000_/RConn3 -- bus399/LConn1
  T_140834620_110000_/RConn1 -- L_140834620/LConn1
  T_140834620_110000_/RConn2 -- L_140834620/LConn2
  L_140834620/LConn3 -- T_140834620_110000_/RConn3 -- bus400/LConn1
  T_200407399__/RConn1 -- L_200407399/LConn1
  T_200407399__/RConn2 -- L_200407399/LConn2
  L_200407399/LConn3 -- T_200407399__/RConn3 -- bus401/LConn1
  T_26329645_110000_/RConn1 -- L_26329645/LConn1
  T_26329645_110000_/RConn2 -- L_26329645/LConn2
  L_26329645/LConn3 -- T_26329645_110000_/RConn3 -- bus402/LConn1
  T_259365224__/RConn1 -- L_259365224/LConn1
  T_259365224__/RConn2 -- L_259365224/LConn2
  L_259365224/LConn3 -- T_259365224__/RConn3 -- bus403/LConn1
  T_158104301_110000_/RConn1 -- L_158104301/LConn1
  T_158104301_110000_/RConn2 -- L_158104301/LConn2
  L_158104301/LConn3 -- T_158104301_110000_/RConn3 -- bus404/LConn1
  T_148312425__/RConn1 -- L_148312425/LConn1
  T_148312425__/RConn2 -- L_148312425/LConn2
  L_148312425/LConn3 -- T_148312425__/RConn3 -- bus405/LConn1
  T_117383986_110000_/RConn1 -- L_117383986/LConn1
  T_117383986_110000_/RConn2 -- L_117383986/LConn2
  L_117383986/LConn3 -- T_117383986_110000_/RConn3 -- bus406/LConn1
  T_355823297__/RConn1 -- L_355823297/LConn1
  T_355823297__/RConn2 -- L_355823297/LConn2
  L_355823297/LConn3 -- T_355823297__/RConn3 -- bus407/LConn1
  T_192143731_110000_/RConn1 -- L_192143731/LConn1
  T_192143731_110000_/RConn2 -- L_192143731/LConn2
  L_192143731/LConn3 -- T_192143731_110000_/RConn3 -- bus408/LConn1
  T_136370548_110000_/RConn1 -- L_136370548/LConn1
  T_136370548_110000_/RConn2 -- L_136370548/LConn2
  L_136370548/LConn3 -- T_136370548_110000_/RConn3 -- bus409/LConn1
  T_162675317__/RConn1 -- L_162675317/LConn1
  T_162675317__/RConn2 -- L_162675317/LConn2
  L_162675317/LConn3 -- T_162675317__/RConn3 -- bus410/LConn1
  T_148596527_110000_/RConn1 -- L_148596527/LConn1
  T_148596527_110000_/RConn2 -- L_148596527/LConn2
  L_148596527/LConn3 -- T_148596527_110000_/RConn3 -- bus411/LConn1
  T_98576761_110000_/RConn1 -- L_98576761/LConn1
  T_98576761_110000_/RConn2 -- L_98576761/LConn2
  L_98576761/LConn3 -- T_98576761_110000_/RConn3 -- bus412/LConn1
  T_217032427__/RConn1 -- L_217032427/LConn1
  T_217032427__/RConn2 -- L_217032427/LConn2
  L_217032427/LConn3 -- T_217032427__/RConn3 -- bus413/LConn1
  T_118766661_110000_/RConn1 -- L_118766661/LConn1
  T_118766661_110000_/RConn2 -- L_118766661/LConn2
  L_118766661/LConn3 -- T_118766661_110000_/RConn3 -- bus414/LConn1
  T_152315970_110000_/RConn1 -- L_152315970/LConn1
  T_152315970_110000_/RConn2 -- L_152315970/LConn2
  L_152315970/LConn3 -- T_152315970_110000_/RConn3 -- bus415/LConn1
  T_97264036__/RConn1 -- L_97264036/LConn1
  T_97264036__/RConn2 -- L_97264036/LConn2
  L_97264036/LConn3 -- T_97264036__/RConn3 -- bus416/LConn1
  T_40101584_110000_/RConn1 -- L_40101584/LConn1
  T_40101584_110000_/RConn2 -- L_40101584/LConn2
  L_40101584/LConn3 -- T_40101584_110000_/RConn3 -- bus417/LConn1
  T_142035550_110000_/RConn1 -- L_142035550/LConn1
  T_142035550_110000_/RConn2 -- L_142035550/LConn2
  L_142035550/LConn3 -- T_142035550_110000_/RConn3 -- bus418/LConn1
  T_182503916_110000_/RConn1 -- L_182503916/LConn1
  T_182503916_110000_/RConn2 -- L_182503916/LConn2
  L_182503916/LConn3 -- T_182503916_110000_/RConn3 -- bus419/LConn1
  T_364224532__/RConn1 -- L_364224532/LConn1
  T_364224532__/RConn2 -- L_364224532/LConn2
  L_364224532/LConn3 -- T_364224532__/RConn3 -- bus420/LConn1
  T_104060546_110000_/RConn1 -- L_104060546/LConn1
  T_104060546_110000_/RConn2 -- L_104060546/LConn2
  L_104060546/LConn3 -- T_104060546_110000_/RConn3 -- bus421/LConn1
  T_166909843_110000_/RConn1 -- L_166909843/LConn1
  T_166909843_110000_/RConn2 -- L_166909843/LConn2
  L_166909843/LConn3 -- T_166909843_110000_/RConn3 -- bus422/LConn1
  T_377338368_110000_/RConn1 -- L_377338368/LConn1
  T_377338368_110000_/RConn2 -- L_377338368/LConn2
  L_377338368/LConn3 -- T_377338368_110000_/RConn3 -- bus423/LConn1
  T_32910454__/RConn1 -- L_32910454/LConn1
  T_32910454__/RConn2 -- L_32910454/LConn2
  L_32910454/LConn3 -- T_32910454__/RConn3 -- bus424/LConn1
  T_168049346_110000_Empower/RConn1 -- L_168049346/LConn1
  T_168049346_110000_Empower/RConn2 -- L_168049346/LConn2
  L_168049346/LConn3 -- T_168049346_110000_Empower/RConn3 -- bus425/LConn1
  T_140677655_110000_/RConn1 -- L_140677655/LConn1
  T_140677655_110000_/RConn2 -- L_140677655/LConn2
  L_140677655/LConn3 -- T_140677655_110000_/RConn3 -- bus426/LConn1
  T_205715364_110000_/RConn1 -- L_205715364/LConn1
  T_205715364_110000_/RConn2 -- L_205715364/LConn2
  L_205715364/LConn3 -- T_205715364_110000_/RConn3 -- bus427/LConn1
  T_142434847_110000_/RConn1 -- L_142434847/LConn1
  T_142434847_110000_/RConn2 -- L_142434847/LConn2
  L_142434847/LConn3 -- T_142434847_110000_/RConn3 -- bus428/LConn1
  T_255787563_110000_/RConn1 -- L_255787563/LConn1
  T_255787563_110000_/RConn2 -- L_255787563/LConn2
  L_255787563/LConn3 -- T_255787563_110000_/RConn3 -- bus429/LConn1
  T_167186210_110000_/RConn1 -- L_167186210/LConn1
  T_167186210_110000_/RConn2 -- L_167186210/LConn2
  L_167186210/LConn3 -- T_167186210_110000_/RConn3 -- bus430/LConn1
  T_151583286_110000_/RConn1 -- L_151583286/LConn1
  T_151583286_110000_/RConn2 -- L_151583286/LConn2
  L_151583286/LConn3 -- T_151583286_110000_/RConn3 -- bus431/LConn1
  T_178307639__/RConn1 -- L_178307639/LConn1
  T_178307639__/RConn2 -- L_178307639/LConn2
  L_178307639/LConn3 -- T_178307639__/RConn3 -- bus432/LConn1
  T_167455825__/RConn1 -- L_167455825/LConn1
  T_167455825__/RConn2 -- L_167455825/LConn2
  L_167455825/LConn3 -- T_167455825__/RConn3 -- bus433/LConn1
  T_348251886_110000_/RConn1 -- L_348251886/LConn1
  T_348251886_110000_/RConn2 -- L_348251886/LConn2
  L_348251886/LConn3 -- T_348251886_110000_/RConn3 -- bus434/LConn1
  T_178639425_110000_/RConn1 -- L_178639425/LConn1
  T_178639425_110000_/RConn2 -- L_178639425/LConn2
  L_178639425/LConn3 -- T_178639425_110000_/RConn3 -- bus435/LConn1
  T_46201634_110000_/RConn1 -- L_46201634/LConn1
  T_46201634_110000_/RConn2 -- L_46201634/LConn2
  L_46201634/LConn3 -- T_46201634_110000_/RConn3 -- bus436/LConn1
  T_178694062__/RConn1 -- L_178694062/LConn1
  T_178694062__/RConn2 -- L_178694062/LConn2
  L_178694062/LConn3 -- T_178694062__/RConn3 -- bus437/LConn1
  T_28258887__/RConn1 -- L_28258887/LConn1
  T_28258887__/RConn2 -- L_28258887/LConn2
  L_28258887/LConn3 -- T_28258887__/RConn3 -- bus438/LConn1
  T_28484367__/RConn1 -- L_28484367/LConn1
  T_28484367__/RConn2 -- L_28484367/LConn2
  L_28484367/LConn3 -- T_28484367__/RConn3 -- bus439/LConn1
  T_88283757_110000_/RConn1 -- L_88283757/LConn1
  T_88283757_110000_/RConn2 -- L_88283757/LConn2
  L_88283757/LConn3 -- T_88283757_110000_/RConn3 -- bus440/LConn1
  T_35263666_110000_/RConn1 -- L_35263666/LConn1
  T_35263666_110000_/RConn2 -- L_35263666/LConn2
  L_35263666/LConn3 -- T_35263666_110000_/RConn3 -- bus441/LConn1
  T_371246420_110000_/RConn1 -- L_371246420/LConn1
  T_371246420_110000_/RConn2 -- L_371246420/LConn2
  L_371246420/LConn3 -- T_371246420_110000_/RConn3 -- bus442/LConn1
  T_93624966_110000_/RConn1 -- L_93624966/LConn1
  T_93624966_110000_/RConn2 -- L_93624966/LConn2
  L_93624966/LConn3 -- T_93624966_110000_/RConn3 -- bus443/LConn1
  T_169018002__/RConn1 -- L_169018002/LConn1
  T_169018002__/RConn2 -- L_169018002/LConn2
  L_169018002/LConn3 -- T_169018002__/RConn3 -- bus444/LConn1
  T_220230343_110000_/RConn1 -- L_220230343/LConn1
  T_220230343_110000_/RConn2 -- L_220230343/LConn2
  L_220230343/LConn3 -- T_220230343_110000_/RConn3 -- bus445/LConn1
  T_220230350_110000_/RConn1 -- L_220230350/LConn1
  T_220230350_110000_/RConn2 -- L_220230350/LConn2
  L_220230350/LConn3 -- T_220230350_110000_/RConn3 -- bus446/LConn1
  T_36977363__/RConn1 -- L_36977363/LConn1
  T_36977363__/RConn2 -- L_36977363/LConn2
  L_36977363/LConn3 -- T_36977363__/RConn3 -- bus447/LConn1
  T_150204241_110000_/RConn1 -- L_150204241/LConn1
  T_150204241_110000_/RConn2 -- L_150204241/LConn2
  L_150204241/LConn3 -- T_150204241_110000_/RConn3 -- bus448/LConn1
  T_94091993_110000_/RConn1 -- L_94091993/LConn1
  T_94091993_110000_/RConn2 -- L_94091993/LConn2
  L_94091993/LConn3 -- T_94091993_110000_/RConn3 -- bus449/LConn1
  T_93582884_110000_/RConn1 -- L_93582884/LConn1
  T_93582884_110000_/RConn2 -- L_93582884/LConn2
  L_93582884/LConn3 -- T_93582884_110000_/RConn3 -- bus450/LConn1
  T_158104293_110000_/RConn1 -- L_158104293/LConn1
  T_158104293_110000_/RConn2 -- L_158104293/LConn2
  L_158104293/LConn3 -- T_158104293_110000_/RConn3 -- bus451/LConn1
  T_319750899_110000;20000_Fortum/RConn1 -- L_319750899/LConn1
  T_319750899_110000;20000_Fortum/RConn2 -- L_319750899/LConn2
  L_319750899/LConn3 -- T_319750899_110000;20000_Fortum/RConn3 -- bus452/LConn1
  T_348349188__/RConn1 -- L_348349188/LConn1
  T_348349188__/RConn2 -- L_348349188/LConn2
  L_348349188/LConn3 -- T_348349188__/RConn3 -- bus453/LConn1
  T_348349190_110000_/RConn1 -- L_348349190/LConn1
  T_348349190_110000_/RConn2 -- L_348349190/LConn2
  L_348349190/LConn3 -- T_348349190_110000_/RConn3 -- bus454/LConn1
  T_153187093_110000_/RConn1 -- L_153187093/LConn1
  T_153187093_110000_/RConn2 -- L_153187093/LConn2
  L_153187093/LConn3 -- T_153187093_110000_/RConn3 -- bus455/LConn1
  T_159935727__/RConn1 -- L_159935727/LConn1
  T_159935727__/RConn2 -- L_159935727/LConn2
  L_159935727/LConn3 -- T_159935727__/RConn3 -- bus456/LConn1
  T_158031219_110000_/RConn1 -- L_158031219/LConn1
  T_158031219_110000_/RConn2 -- L_158031219/LConn2
  L_158031219/LConn3 -- T_158031219_110000_/RConn3 -- bus457/LConn1
  T_26391332__Pitajanmaki/RConn1 -- L_26391332/LConn1
  T_26391332__Pitajanmaki/RConn2 -- L_26391332/LConn2
  L_26391332/LConn3 -- T_26391332__Pitajanmaki/RConn3 -- bus458/LConn1
  T_26367884_110000_/RConn1 -- L_26367884/LConn1
  T_26367884_110000_/RConn2 -- L_26367884/LConn2
  L_26367884/LConn3 -- T_26367884_110000_/RConn3 -- bus459/LConn1
  T_197245741_110000_/RConn1 -- L_197245741/LConn1
  T_197245741_110000_/RConn2 -- L_197245741/LConn2
  L_197245741/LConn3 -- T_197245741_110000_/RConn3 -- bus460/LConn1
  T_153576520_110000_/RConn1 -- L_153576520/LConn1
  T_153576520_110000_/RConn2 -- L_153576520/LConn2
  L_153576520/LConn3 -- T_153576520_110000_/RConn3 -- bus461/LConn1
  T_137112425_110000_/RConn1 -- L_137112425/LConn1
  T_137112425_110000_/RConn2 -- L_137112425/LConn2
  L_137112425/LConn3 -- T_137112425_110000_/RConn3 -- bus462/LConn1
  T_132652863__/RConn1 -- L_132652863/LConn1
  T_132652863__/RConn2 -- L_132652863/LConn2
  L_132652863/LConn3 -- T_132652863__/RConn3 -- bus463/LConn1
  T_136355274_110000_/RConn1 -- L_136355274/LConn1
  T_136355274_110000_/RConn2 -- L_136355274/LConn2
  L_136355274/LConn3 -- T_136355274_110000_/RConn3 -- bus464/LConn1
  T_211471223_110000_/RConn1 -- L_211471223/LConn1
  T_211471223_110000_/RConn2 -- L_211471223/LConn2
  L_211471223/LConn3 -- T_211471223_110000_/RConn3 -- bus465/LConn1
  T_129112047_110000_/RConn1 -- L_129112047/LConn1
  T_129112047_110000_/RConn2 -- L_129112047/LConn2
  L_129112047/LConn3 -- T_129112047_110000_/RConn3 -- bus466/LConn1
  T_155899286_110000_/RConn1 -- L_155899286/LConn1
  T_155899286_110000_/RConn2 -- L_155899286/LConn2
  L_155899286/LConn3 -- T_155899286_110000_/RConn3 -- bus467/LConn1
  T_94667682_110000_/RConn1 -- L_94667682/LConn1
  T_94667682_110000_/RConn2 -- L_94667682/LConn2
  L_94667682/LConn3 -- T_94667682_110000_/RConn3 -- bus468/LConn1
  T_95184246_110000_/RConn1 -- L_95184246/LConn1
  T_95184246_110000_/RConn2 -- L_95184246/LConn2
  L_95184246/LConn3 -- T_95184246_110000_/RConn3 -- bus469/LConn1
  T_142846911__/RConn1 -- L_142846911/LConn1
  T_142846911__/RConn2 -- L_142846911/LConn2
  L_142846911/LConn3 -- T_142846911__/RConn3 -- bus470/LConn1
  T_200166363__/RConn1 -- L_200166363/LConn1
  T_200166363__/RConn2 -- L_200166363/LConn2
  L_200166363/LConn3 -- T_200166363__/RConn3 -- bus471/LConn1
  T_400589797_110000_/RConn1 -- L_400589797/LConn1
  T_400589797_110000_/RConn2 -- L_400589797/LConn2
  L_400589797/LConn3 -- T_400589797_110000_/RConn3 -- bus472/LConn1
  T_400588215_110000_/RConn1 -- L_400588215/LConn1
  T_400588215_110000_/RConn2 -- L_400588215/LConn2
  L_400588215/LConn3 -- T_400588215_110000_/RConn3 -- bus473/LConn1
  T_92656655_110000_/RConn1 -- L_92656655/LConn1
  T_92656655_110000_/RConn2 -- L_92656655/LConn2
  L_92656655/LConn3 -- T_92656655_110000_/RConn3 -- bus474/LConn1
  T_174266079__/RConn1 -- L_174266079/LConn1
  T_174266079__/RConn2 -- L_174266079/LConn2
  L_174266079/LConn3 -- T_174266079__/RConn3 -- bus475/LConn1
  T_363802508_110000_/RConn1 -- L_363802508/LConn1
  T_363802508_110000_/RConn2 -- L_363802508/LConn2
  L_363802508/LConn3 -- T_363802508_110000_/RConn3 -- bus476/LConn1
  T_98393115_110000_/RConn1 -- L_98393115/LConn1
  T_98393115_110000_/RConn2 -- L_98393115/LConn2
  L_98393115/LConn3 -- T_98393115_110000_/RConn3 -- bus477/LConn1
  T_391142037_110000_/RConn1 -- L_391142037/LConn1
  T_391142037_110000_/RConn2 -- L_391142037/LConn2
  L_391142037/LConn3 -- T_391142037_110000_/RConn3 -- bus478/LConn1
  T_122703556__/RConn1 -- L_122703556/LConn1
  T_122703556__/RConn2 -- L_122703556/LConn2
  L_122703556/LConn3 -- T_122703556__/RConn3 -- bus479/LConn1
  T_285201507__/RConn1 -- L_285201507/LConn1
  T_285201507__/RConn2 -- L_285201507/LConn2
  L_285201507/LConn3 -- T_285201507__/RConn3 -- bus480/LConn1
  T_235817994_110000_/RConn1 -- L_235817994/LConn1
  T_235817994_110000_/RConn2 -- L_235817994/LConn2
  L_235817994/LConn3 -- T_235817994_110000_/RConn3 -- bus481/LConn1
  T_89956002_110000_/RConn1 -- L_89956002/LConn1
  T_89956002_110000_/RConn2 -- L_89956002/LConn2
  L_89956002/LConn3 -- T_89956002_110000_/RConn3 -- bus482/LConn1
  T_88020737_110000_/RConn1 -- L_88020737/LConn1
  T_88020737_110000_/RConn2 -- L_88020737/LConn2
  L_88020737/LConn3 -- T_88020737_110000_/RConn3 -- bus483/LConn1
  T_88020687_110000_/RConn1 -- L_88020687/LConn1
  T_88020687_110000_/RConn2 -- L_88020687/LConn2
  L_88020687/LConn3 -- T_88020687_110000_/RConn3 -- bus484/LConn1
  T_345672987_110000_/RConn1 -- L_345672987/LConn1
  T_345672987_110000_/RConn2 -- L_345672987/LConn2
  L_345672987/LConn3 -- T_345672987_110000_/RConn3 -- bus485/LConn1
  T_30483473__/RConn1 -- L_30483473/LConn1
  T_30483473__/RConn2 -- L_30483473/LConn2
  L_30483473/LConn3 -- T_30483473__/RConn3 -- bus486/LConn1
  T_218734234__/RConn1 -- L_218734234/LConn1
  T_218734234__/RConn2 -- L_218734234/LConn2
  L_218734234/LConn3 -- T_218734234__/RConn3 -- bus487/LConn1
  T_167705754_110000_/RConn1 -- L_167705754/LConn1
  T_167705754_110000_/RConn2 -- L_167705754/LConn2
  L_167705754/LConn3 -- T_167705754_110000_/RConn3 -- bus488/LConn1
  T_122838157_110000_/RConn1 -- L_122838157/LConn1
  T_122838157_110000_/RConn2 -- L_122838157/LConn2
  L_122838157/LConn3 -- T_122838157_110000_/RConn3 -- bus489/LConn1
  T_140227959_110000_/RConn1 -- L_140227959/LConn1
  T_140227959_110000_/RConn2 -- L_140227959/LConn2
  L_140227959/LConn3 -- T_140227959_110000_/RConn3 -- bus490/LConn1
  T_167862173__/RConn1 -- L_167862173/LConn1
  T_167862173__/RConn2 -- L_167862173/LConn2
  L_167862173/LConn3 -- T_167862173__/RConn3 -- bus491/LConn1
  T_345672928__/RConn1 -- L_345672928/LConn1
  T_345672928__/RConn2 -- L_345672928/LConn2
  L_345672928/LConn3 -- T_345672928__/RConn3 -- bus492/LConn1
  T_348349199_110000_/RConn1 -- L_348349199/LConn1
  T_348349199_110000_/RConn2 -- L_348349199/LConn2
  L_348349199/LConn3 -- T_348349199_110000_/RConn3 -- bus493/LConn1
  T_162950429_110000_/RConn1 -- L_162950429/LConn1
  T_162950429_110000_/RConn2 -- L_162950429/LConn2
  L_162950429/LConn3 -- T_162950429_110000_/RConn3 -- bus494/LConn1
  T_162690719_110000_/RConn1 -- L_162690719/LConn1
  T_162690719_110000_/RConn2 -- L_162690719/LConn2
  L_162690719/LConn3 -- T_162690719_110000_/RConn3 -- bus495/LConn1
  T_252609822_110000_/RConn1 -- L_252609822/LConn1
  T_252609822_110000_/RConn2 -- L_252609822/LConn2
  L_252609822/LConn3 -- T_252609822_110000_/RConn3 -- bus496/LConn1
  T_158219552_110000_/RConn1 -- L_158219552/LConn1
  T_158219552_110000_/RConn2 -- L_158219552/LConn2
  L_158219552/LConn3 -- T_158219552_110000_/RConn3 -- bus497/LConn1
  T_149818659_110000_/RConn1 -- L_149818659/LConn1
  T_149818659_110000_/RConn2 -- L_149818659/LConn2
  L_149818659/LConn3 -- T_149818659_110000_/RConn3 -- bus498/LConn1
  T_165373253_110000_/RConn1 -- L_165373253/LConn1
  T_165373253_110000_/RConn2 -- L_165373253/LConn2
  L_165373253/LConn3 -- T_165373253_110000_/RConn3 -- bus499/LConn1
  T_130069830__/RConn1 -- L_130069830/LConn1
  T_130069830__/RConn2 -- L_130069830/LConn2
  L_130069830/LConn3 -- T_130069830__/RConn3 -- bus500/LConn1
  T_130069831_110000_/RConn1 -- L_130069831/LConn1
  T_130069831_110000_/RConn2 -- L_130069831/LConn2
  L_130069831/LConn3 -- T_130069831_110000_/RConn3 -- bus501/LConn1
  T_130069833_110000_/RConn1 -- L_130069833/LConn1
  T_130069833_110000_/RConn2 -- L_130069833/LConn2
  L_130069833/LConn3 -- T_130069833_110000_/RConn3 -- bus502/LConn1
  T_147699112__/RConn1 -- L_147699112/LConn1
  T_147699112__/RConn2 -- L_147699112/LConn2
  L_147699112/LConn3 -- T_147699112__/RConn3 -- bus503/LConn1
  T_147699118_110000_/RConn1 -- L_147699118/LConn1
  T_147699118_110000_/RConn2 -- L_147699118/LConn2
  L_147699118/LConn3 -- T_147699118_110000_/RConn3 -- bus504/LConn1
  T_178234889_110000_/RConn1 -- L_178234889/LConn1
  T_178234889_110000_/RConn2 -- L_178234889/LConn2
  L_178234889/LConn3 -- T_178234889_110000_/RConn3 -- bus505/LConn1
  T_178234890_110000_/RConn1 -- L_178234890/LConn1
  T_178234890_110000_/RConn2 -- L_178234890/LConn2
  L_178234890/LConn3 -- T_178234890_110000_/RConn3 -- bus506/LConn1
  T_136361669_110000_/RConn1 -- L_136361669/LConn1
  T_136361669_110000_/RConn2 -- L_136361669/LConn2
  L_136361669/LConn3 -- T_136361669_110000_/RConn3 -- bus507/LConn1
  T_159172094_110000_/RConn1 -- L_159172094/LConn1
  T_159172094_110000_/RConn2 -- L_159172094/LConn2
  L_159172094/LConn3 -- T_159172094_110000_/RConn3 -- bus508/LConn1
  T_104410725__/RConn1 -- L_104410725/LConn1
  T_104410725__/RConn2 -- L_104410725/LConn2
  L_104410725/LConn3 -- T_104410725__/RConn3 -- bus509/LConn1
  T_178181897_110000_/RConn1 -- L_178181897/LConn1
  T_178181897_110000_/RConn2 -- L_178181897/LConn2
  L_178181897/LConn3 -- T_178181897_110000_/RConn3 -- bus510/LConn1
  T_198362738_110000_/RConn1 -- L_198362738/LConn1
  T_198362738_110000_/RConn2 -- L_198362738/LConn2
  L_198362738/LConn3 -- T_198362738_110000_/RConn3 -- bus511/LConn1
  T_198362740_110000_/RConn1 -- L_198362740/LConn1
  T_198362740_110000_/RConn2 -- L_198362740/LConn2
  L_198362740/LConn3 -- T_198362740_110000_/RConn3 -- bus512/LConn1
  T_198362741_110000_/RConn1 -- L_198362741/LConn1
  T_198362741_110000_/RConn2 -- L_198362741/LConn2
  L_198362741/LConn3 -- T_198362741_110000_/RConn3 -- bus513/LConn1
  T_143511169_110000_/RConn1 -- L_143511169/LConn1
  T_143511169_110000_/RConn2 -- L_143511169/LConn2
  L_143511169/LConn3 -- T_143511169_110000_/RConn3 -- bus514/LConn1
  T_143511171_110000_/RConn1 -- L_143511171/LConn1
  T_143511171_110000_/RConn2 -- L_143511171/LConn2
  L_143511171/LConn3 -- T_143511171_110000_/RConn3 -- bus515/LConn1
  T_26330814_110000_/RConn1 -- L_26330814/LConn1
  T_26330814_110000_/RConn2 -- L_26330814/LConn2
  L_26330814/LConn3 -- T_26330814_110000_/RConn3 -- bus516/LConn1
  T_53047221_110000_/RConn1 -- L_53047221/LConn1
  T_53047221_110000_/RConn2 -- L_53047221/LConn2
  L_53047221/LConn3 -- T_53047221_110000_/RConn3 -- bus517/LConn1
  T_136361666_110000_/RConn1 -- L_136361666/LConn1
  T_136361666_110000_/RConn2 -- L_136361666/LConn2
  L_136361666/LConn3 -- T_136361666_110000_/RConn3 -- bus518/LConn1
  T_87670542_110000_/RConn1 -- L_87670542/LConn1
  T_87670542_110000_/RConn2 -- L_87670542/LConn2
  L_87670542/LConn3 -- T_87670542_110000_/RConn3 -- bus519/LConn1
  T_177676064__/RConn1 -- L_177676064/LConn1
  T_177676064__/RConn2 -- L_177676064/LConn2
  L_177676064/LConn3 -- T_177676064__/RConn3 -- bus520/LConn1
  T_167176159_110000_/RConn1 -- L_167176159/LConn1
  T_167176159_110000_/RConn2 -- L_167176159/LConn2
  L_167176159/LConn3 -- T_167176159_110000_/RConn3 -- bus521/LConn1
  T_167184034__/RConn1 -- L_167184034/LConn1
  T_167184034__/RConn2 -- L_167184034/LConn2
  L_167184034/LConn3 -- T_167184034__/RConn3 -- bus522/LConn1
  T_400582573_110000_/RConn1 -- L_400582573/LConn1
  T_400582573_110000_/RConn2 -- L_400582573/LConn2
  L_400582573/LConn3 -- T_400582573_110000_/RConn3 -- bus523/LConn1
  T_400582583_110000_/RConn1 -- L_400582583/LConn1
  T_400582583_110000_/RConn2 -- L_400582583/LConn2
  L_400582583/LConn3 -- T_400582583_110000_/RConn3 -- bus524/LConn1
  T_391140226_400000_/RConn1 -- L_391140226/LConn1
  T_391140226_400000_/RConn2 -- L_391140226/LConn2
  L_391140226/LConn3 -- T_391140226_400000_/RConn3 -- bus525/LConn1
  T_149965733_400000;220000_/RConn1 -- L_149965733/LConn1
  T_149965733_400000;220000_/RConn2 -- L_149965733/LConn2
  L_149965733/LConn3 -- T_149965733_400000;220000_/RConn3 -- bus526/LConn1
  T_239242345_400000_/RConn1 -- L_239242345/LConn1
  T_239242345_400000_/RConn2 -- L_239242345/LConn2
  L_239242345/LConn3 -- T_239242345_400000_/RConn3 -- bus527/LConn1
  T_53047196_400000_/RConn1 -- L_53047196/LConn1
  T_53047196_400000_/RConn2 -- L_53047196/LConn2
  L_53047196/LConn3 -- T_53047196_400000_/RConn3 -- bus528/LConn1
  T_98589905_400000_/RConn1 -- L_98589905/LConn1
  T_98589905_400000_/RConn2 -- L_98589905/LConn2
  L_98589905/LConn3 -- T_98589905_400000_/RConn3 -- bus529/LConn1
  T_286955409_400000_Petäjäskoski/RConn1 -- L_286955409/LConn1
  T_286955409_400000_Petäjäskoski/RConn2 -- L_286955409/LConn2
  L_286955409/LConn3 -- T_286955409_400000_Petäjäskoski/RConn3 -- bus530/LConn1
  T_348358044_400000;110000_/RConn1 -- L_348358044/LConn1
  T_348358044_400000;110000_/RConn2 -- L_348358044/LConn2
  L_348358044/LConn3 -- T_348358044_400000;110000_/RConn3 -- bus531/LConn1
  T_98554218__/RConn1 -- L_98554218/LConn1
  T_98554218__/RConn2 -- L_98554218/LConn2
  L_98554218/LConn3 -- T_98554218__/RConn3 -- bus532/LConn1
  T_98609844_400000_/RConn1 -- L_98609844/LConn1
  T_98609844_400000_/RConn2 -- L_98609844/LConn2
  L_98609844/LConn3 -- T_98609844_400000_/RConn3 -- bus533/LConn1
  T_217032425_400000_/RConn1 -- L_217032425/LConn1
  T_217032425_400000_/RConn2 -- L_217032425/LConn2
  L_217032425/LConn3 -- T_217032425_400000_/RConn3 -- bus534/LConn1
